simulink model "Dinamica5seg"  (R2021b)
settings: Solver=VariableStepAuto  StartTime=0.0  StopTime=70  RelTol=1e-3
(part 2 of 3)

== matlab function Dinamica5seg/ROBOT ==
  data: q1 input; tao1 output; tao2 output; tao3 output; dq1 input; d2q1 input; q2 input; dq2 input; d2q2 input; q3 input; dq3 input; d2q3 input; q4 input; dq4 input; d2q4 input; m1 input; m2 input; m3 input; m4 input; l1 input; l2 input; l3 input; l4 input; g input; tao4 output
function [tao1, tao2, tao3, tao4] = EulerLagrange(q1, dq1, d2q1, q2, dq2, d2q2, q3, dq3, d2q3, q4, dq4, d2q4, m1, m2, m3, m4, l1, l2, l3, l4, g)
%tao1= (40812255641599999*d2q1)/16777216 - 999120000*dq2^2*cos(q1)^2 + 382320000*dq3^2*cos(q1)^2 + 191160000*dq3^2*cos(q2)^2 - 120720000*dq4^2*cos(q2)^2 + 120720000*dq4^2*cos(q3)^2 + (52562346639359997*dq2^2*sin(2*q1))/67108864 - (4500767812266667*dq3^2*sin(2*q1))/67108864 + 233160000*d2q2*cos(q1) + (9002430409386667*d2q3*cos(q2))/16777216 + 499560000*dq2^2 - 191160000*dq3^2 - (13504093006506667*dq2*dq3*sin(q2))/33554432 + 80480000*d2q4*cos(q1)*cos(q3) - 382320000*dq3^2*cos(q1)^2*cos(q2)^2 + 241440000*dq4^2*cos(q1)^2*cos(q2)^2 - 241440000*dq4^2*cos(q1)^2*cos(q3)^2 + 120720000*dq4^2*cos(q2)^2*cos(q3)^2 + 150920000*d2q3*sin(q1)*sin(q2) + (5850998155946667*d2q4*sin(q2)*sin(q3))/16777216 + d2q1*l1^2*m1 + (d2q1*l1^2*m2)/2 + (d2q1*l1^2*m3)/2 + (d2q1*l1^2*m4)/2 + (d2q1*l3^2*m3)/8 + (d2q1*l3^2*m4)/2 + (d2q1*l4^2*m4)/8 + 241440000*dq2*dq4*cos(q3) + (4500767812266667*dq3^2*cos(q1)*cos(q2)^2*sin(q1))/33554432 - (4500767812266667*dq4^2*cos(q1)*cos(q2)^2*sin(q1))/33554432 + (4500767812266667*dq4^2*cos(q1)*cos(q3)^2*sin(q1))/33554432 + (d2q1*l2^2*m2*cos(q2)^2)/8 + (d2q1*l2^2*m3*cos(q2)^2)/2 + (d2q1*l2^2*m4*cos(q2)^2)/2 - (d2q1*l3^2*m3*cos(q3)^2)/8 - (d2q1*l3^2*m4*cos(q3)^2)/2 - (d2q1*l4^2*m4*cos(q2)^2)/8 - 482880000*dq2*dq4*cos(q1)^2*cos(q3) - (4500767812266667*dq2*dq3*cos(q1)^2*sin(q2))/16777216 - 80480000*d2q4*cos(q2)*sin(q1)*sin(q3) + (g*l1*m1*cos(q1))/2 + g*l1*m2*cos(q1) + g*l1*m3*cos(q1) + g*l1*m4*cos(q1) - 150920000*dq3^2*cos(q1)*cos(q2)*sin(q2) + 80480000*dq4^2*cos(q1)*cos(q2)*sin(q2) - (4500767812266667*dq4^2*cos(q2)*cos(q3)*sin(q3))/33554432 - 241440000*dq4^2*cos(q1)^2*cos(q2)^2*cos(q3)^2 + (d2q3*l3^2*m3*cos(q2))/8 + (d2q3*l3^2*m4*cos(q2))/2 + 301840000*dq2*dq3*cos(q2)*sin(q1) + (7201228499626667*dq2*dq4*cos(q2)*sin(q3))/33554432 - 160960000*dq3*dq4*cos(q1)*sin(q3) + (16202764124160001*dq3*dq4*cos(q3)*sin(q2))/33554432 + (d2q3*l4^2*m4*cos(q2)*cos(q4)^2)/8 + (4500767812266667*dq2*dq4*cos(q1)^2*cos(q2)*sin(q3))/16777216 + 160960000*dq3*dq4*cos(q1)*cos(q2)^2*sin(q3) - (4500767812266667*dq3*dq4*cos(q1)^2*cos(q3)*sin(q2))/16777216 + (4500767812266667*dq4^2*cos(q1)*cos(q2)^2*cos(q3)^2*sin(q1))/33554432 - (dq2*dq3*l3^2*m3*sin(q2))/4 - dq2*dq3*l3^2*m4*sin(q2) + (g*l2*m2*cos(q1)*cos(q2))/2 + g*l2*m3*cos(q1)*cos(q2) + g*l2*m4*cos(q1)*cos(q2) - (dq3^2*l1*l3*m3*sin(q3))/4 - (dq3^2*l1*l3*m4*sin(q3))/2 + (d2q1*l3^2*m3*cos(q2)^2*cos(q3)^2)/8 + (d2q1*l3^2*m4*cos(q2)^2*cos(q3)^2)/2 + (d2q1*l4^2*m4*cos(q2)^2*cos(q4)^2)/8 - (d2q1*l4^2*m4*cos(q3)^2*cos(q4)^2)/8 - (g*l3*m3*sin(q1)*sin(q3))/2 - g*l3*m4*sin(q1)*sin(q3) - (dq1*dq2*l2^2*m2*sin(2*q2))/8 - (dq1*dq2*l2^2*m3*sin(2*q2))/2 - (dq1*dq2*l2^2*m4*sin(2*q2))/2 + (dq1*dq2*l4^2*m4*sin(2*q2))/8 + (dq1*dq3*l3^2*m3*sin(2*q3))/8 + (dq1*dq3*l3^2*m4*sin(2*q3))/2 + 80480000*dq4^2*cos(q3)*sin(q1)*sin(q2)*sin(q3) + (4500767812266667*dq2*dq4*cos(q1)*cos(q3)*sin(q1))/16777216 + (d2q4*l4^2*m4*sin(q2)*sin(q3))/8 - 764640000*dq2*dq3*cos(q1)*sin(q1)*sin(q2) + 241440000*dq3*dq4*cos(q2)*sin(q2)*sin(q3) + 160960000*dq2*dq4*sin(q1)*sin(q2)*sin(q3) + (d2q1*l1*l2*m2*cos(q2))/2 + d2q1*l1*l2*m3*cos(q2) + d2q1*l1*l2*m4*cos(q2) + (d2q3*l1*l3*m3*cos(q3))/4 + (d2q3*l1*l3*m4*cos(q3))/2 + (d2q1*l3*l4*m4*cos(q4))/2 - 80480000*dq4^2*cos(q1)*cos(q2)*cos(q3)^2*sin(q2) + (4500767812266667*dq4^2*cos(q1)^2*cos(q2)*cos(q3)*sin(q3))/16777216 + (d2q1*l2*l3*m3*cos(q2)^2*cos(q3))/2 + d2q1*l2*l3*m4*cos(q2)^2*cos(q3) - (d2q1*l3*l4*m4*cos(q3)^2*cos(q4))/2 + (dq3*dq4*l4^2*m4*cos(q3)*sin(q2))/4 + (g*l3*m3*cos(q1)*cos(q2)*cos(q3))/2 + g*l3*m4*cos(q1)*cos(q2)*cos(q3) + (dq2^2*l2*l3*m3*cos(q2)*sin(q3))/4 + (dq2^2*l2*l3*m4*cos(q2)*sin(q3))/2 - (dq3^2*l2*l3*m3*cos(q2)*sin(q3))/4 - (dq3^2*l2*l3*m4*cos(q2)*sin(q3))/2 - (dq3^2*l1*l4*m4*cos(q4)*sin(q3))/4 - (dq4^2*l1*l4*m4*cos(q4)*sin(q3))/4 - (g*l4*m4*cos(q1)*sin(q2)*sin(q4))/2 - (g*l4*m4*cos(q4)*sin(q1)*sin(q3))/2 - (dq1*dq2*l1*l2*m2*sin(q2))/2 - dq1*dq2*l1*l2*m3*sin(q2) - dq1*dq2*l1*l2*m4*sin(q2) + (dq1*dq2*l2*l4*m4*sin(q4))/2 - (dq1*dq4*l3*l4*m4*sin(q4))/2 + 482880000*dq4^2*cos(q1)*cos(q2)*cos(q3)*sin(q1)*sin(q3) + (dq2*dq3*l3^2*m3*cos(q3)^2*sin(q2))/4 + dq2*dq3*l3^2*m4*cos(q3)^2*sin(q2) - (dq2*dq3*l4^2*m4*cos(q4)^2*sin(q2))/4 + (d2q1*l4^2*m4*cos(q2)^2*cos(q3)^2*cos(q4)^2)/8 + (d2q2*l3^2*m3*cos(q3)*sin(q2)*sin(q3))/8 + (d2q2*l3^2*m4*cos(q3)*sin(q2)*sin(q3))/2 + 482880000*dq2*dq4*cos(q1)*cos(q2)*sin(q1)*sin(q3) - 482880000*dq3*dq4*cos(q1)*cos(q3)*sin(q1)*sin(q2) + (d2q1*l1*l3*m3*cos(q2)*cos(q3))/2 + d2q1*l1*l3*m4*cos(q2)*cos(q3) + (d2q3*l2*l3*m3*cos(q2)*cos(q3))/4 + (d2q3*l2*l3*m4*cos(q2)*cos(q3))/2 + (d2q3*l1*l4*m4*cos(q3)*cos(q4))/4 + (d2q3*l3*l4*m4*cos(q2)*cos(q4))/2 + (d2q2*l2*l3*m3*sin(q2)*sin(q3))/4 - (d2q1*l1*l4*m4*sin(q2)*sin(q4))/2 + (d2q2*l2*l3*m4*sin(q2)*sin(q3))/2 - (d2q4*l1*l4*m4*sin(q3)*sin(q4))/4 + (dq2^2*l3^2*m3*cos(q2)*cos(q3)*sin(q3))/8 + (dq2^2*l3^2*m4*cos(q2)*cos(q3)*sin(q3))/2 - 482880000*dq3*dq4*cos(q1)^2*cos(q2)*sin(q2)*sin(q3) - (dq2^2*l3*l4*m4*sin(q2)*sin(q3)*sin(q4))/4 + (dq3^2*l3*l4*m4*sin(q2)*sin(q3)*sin(q4))/4 - (dq4^2*l3*l4*m4*sin(q2)*sin(q3)*sin(q4))/4 + (dq2^2*l4^2*m4*cos(q2)*cos(q3)*cos(q4)^2*sin(q3))/8 - (dq1*dq2*l1*l3*m3*cos(q3)*sin(q2))/2 - dq1*dq2*l1*l3*m4*cos(q3)*sin(q2) - (dq1*dq3*l1*l3*m3*cos(q2)*sin(q3))/2 - dq1*dq3*l1*l3*m4*cos(q2)*sin(q3) - (dq1*dq2*l1*l4*m4*cos(q2)*sin(q4))/2 - (dq1*dq4*l1*l4*m4*cos(q4)*sin(q2))/2 + (dq1*dq2*l3*l4*m4*cos(q3)*sin(q4))/2 - dq2*dq3*l3*l4*m4*cos(q4)*sin(q2) - (dq3*dq4*l1*l4*m4*cos(q3)*sin(q4))/2 - (dq3*dq4*l3*l4*m4*cos(q2)*sin(q4))/2 + (d2q1*l3*l4*m4*cos(q2)^2*cos(q3)^2*cos(q4))/2 - (dq1*dq2*l3^2*m3*cos(q2)*cos(q3)^2*sin(q2))/4 - dq1*dq2*l3^2*m4*cos(q2)*cos(q3)^2*sin(q2) - (dq1*dq3*l3^2*m3*cos(q2)^2*cos(q3)*sin(q3))/4 - (dq1*dq2*l4^2*m4*cos(q2)*cos(q4)^2*sin(q2))/4 - dq1*dq3*l3^2*m4*cos(q2)^2*cos(q3)*sin(q3) + (dq1*dq3*l4^2*m4*cos(q3)*cos(q4)^2*sin(q3))/4 - (dq1*dq4*l4^2*m4*cos(q2)^2*cos(q4)*sin(q4))/4 + (dq2*dq4*l4^2*m4*cos(q2)*cos(q4)^2*sin(q3))/4 + (dq1*dq4*l4^2*m4*cos(q3)^2*cos(q4)*sin(q4))/4 - (dq3*dq4*l4^2*m4*cos(q3)*cos(q4)^2*sin(q2))/4 + (d2q2*l4^2*m4*cos(q2)*cos(q4)*sin(q3)*sin(q4))/8 - (d2q3*l4^2*m4*cos(q3)*cos(q4)*sin(q2)*sin(q4))/8 + (4500767812266667*dq3*dq4*cos(q1)*cos(q2)*sin(q1)*sin(q2)*sin(q3))/16777216 - (dq1*dq3*l2*l3*m3*cos(q2)^2*sin(q3))/2 - dq1*dq3*l2*l3*m4*cos(q2)^2*sin(q3) - dq1*dq2*l2*l4*m4*cos(q2)^2*sin(q4) + (dq1*dq4*l3*l4*m4*cos(q3)^2*sin(q4))/2 + (d2q1*l1*l4*m4*cos(q2)*cos(q3)*cos(q4))/2 + (d2q3*l2*l4*m4*cos(q2)*cos(q3)*cos(q4))/4 - (d2q1*l2*l4*m4*cos(q2)*sin(q2)*sin(q4))/2 + (d2q2*l2*l4*m4*cos(q4)*sin(q2)*sin(q3))/4 + (d2q2*l3*l4*m4*cos(q2)*sin(q3)*sin(q4))/4 - (d2q3*l3*l4*m4*cos(q3)*sin(q2)*sin(q4))/4 - (d2q4*l2*l4*m4*cos(q2)*sin(q3)*sin(q4))/4 + (d2q4*l3*l4*m4*cos(q4)*sin(q2)*sin(q3))/4 + (dq2*dq3*l4^2*m4*cos(q3)^2*cos(q4)^2*sin(q2))/4 + (d2q2*l4^2*m4*cos(q3)*cos(q4)^2*sin(q2)*sin(q3))/8 - (dq2^2*l4^2*m4*cos(q4)*sin(q2)*sin(q3)*sin(q4))/8 + (dq3^2*l4^2*m4*cos(q4)*sin(q2)*sin(q3)*sin(q4))/8 + (d2q1*l2*l4*m4*cos(q2)^2*cos(q3)*cos(q4))/2 + (dq1*dq4*l4^2*m4*cos(q2)*cos(q3)*sin(q2))/4 + (dq1*dq2*l4^2*m4*cos(q3)*cos(q4)*sin(q4))/4 - (dq3*dq4*l4^2*m4*cos(q2)*cos(q4)*sin(q4))/4 + (g*l4*m4*cos(q1)*cos(q2)*cos(q3)*cos(q4))/2 + (dq2^2*l2*l4*m4*cos(q2)*cos(q4)*sin(q3))/4 - (dq3^2*l2*l4*m4*cos(q2)*cos(q4)*sin(q3))/4 - (dq4^2*l2*l4*m4*cos(q2)*cos(q4)*sin(q3))/4 - (dq1*dq2*l4^2*m4*cos(q2)^2*cos(q3)*cos(q4)*sin(q4))/2 - (dq1*dq4*l4^2*m4*cos(q2)*cos(q3)*cos(q4)^2*sin(q2))/2 - (d2q1*l4^2*m4*cos(q2)*cos(q3)*cos(q4)*sin(q2)*sin(q4))/4 - dq1*dq2*l3*l4*m4*cos(q2)^2*cos(q3)*sin(q4) - (dq1*dq3*l2*l4*m4*cos(q2)^2*cos(q4)*sin(q3))/2 - (dq1*dq4*l2*l4*m4*cos(q2)^2*cos(q3)*sin(q4))/2 + dq2*dq3*l3*l4*m4*cos(q3)^2*cos(q4)*sin(q2) - (d2q1*l3*l4*m4*cos(q2)*cos(q3)*sin(q2)*sin(q4))/2 + (d2q2*l3*l4*m4*cos(q3)*cos(q4)*sin(q2)*sin(q3))/2 - (dq1*dq2*l4^2*m4*cos(q2)*cos(q3)^2*cos(q4)^2*sin(q2))/4 - (dq1*dq3*l4^2*m4*cos(q2)^2*cos(q3)*cos(q4)^2*sin(q3))/4 - (dq1*dq4*l4^2*m4*cos(q2)^2*cos(q3)^2*cos(q4)*sin(q4))/4 - (dq1*dq4*l3*l4*m4*cos(q2)^2*cos(q3)^2*sin(q4))/2 + (dq2^2*l3*l4*m4*cos(q2)*cos(q3)*cos(q4)*sin(q3))/2 - dq1*dq2*l2*l3*m3*cos(q2)*cos(q3)*sin(q2) - 2*dq1*dq2*l2*l3*m4*cos(q2)*cos(q3)*sin(q2) - (dq1*dq2*l1*l4*m4*cos(q3)*cos(q4)*sin(q2))/2 - (dq1*dq3*l1*l4*m4*cos(q2)*cos(q4)*sin(q3))/2 - (dq1*dq4*l1*l4*m4*cos(q2)*cos(q3)*sin(q4))/2 - (dq1*dq4*l2*l4*m4*cos(q2)*cos(q4)*sin(q2))/2 + dq1*dq3*l3*l4*m4*cos(q3)*cos(q4)*sin(q3) + (dq2*dq4*l3*l4*m4*cos(q2)*cos(q4)*sin(q3))/2 - (dq3*dq4*l2*l4*m4*cos(q2)*cos(q3)*sin(q4))/2 - dq1*dq2*l3*l4*m4*cos(q2)*cos(q3)^2*cos(q4)*sin(q2) - dq1*dq3*l3*l4*m4*cos(q2)^2*cos(q3)*cos(q4)*sin(q3) + (dq1*dq3*l4^2*m4*cos(q2)*cos(q4)*sin(q2)*sin(q3)*sin(q4))/4 - (dq2*dq4*l4^2*m4*cos(q3)*cos(q4)*sin(q2)*sin(q3)*sin(q4))/4 - dq1*dq2*l2*l4*m4*cos(q2)*cos(q3)*cos(q4)*sin(q2) - (dq1*dq4*l3*l4*m4*cos(q2)*cos(q3)*cos(q4)*sin(q2))/2 + (dq1*dq3*l3*l4*m4*cos(q2)*sin(q2)*sin(q3)*sin(q4))/2 - (dq2*dq4*l3*l4*m4*cos(q3)*sin(q2)*sin(q3)*sin(q4))/2;
%tao2= (20862803640320001*d2q2)/33554432 + 499560000*d2q2*sin(2*q1) - 233160000*dq1^2*sin(q1) + 150920000*dq3^2*sin(q1) - 80480000*dq4^2*sin(q1) - 999120000*dq1*dq2 + 233160000*d2q1*cos(q1) + (7201228499626667*d2q4*cos(q3))/33554432 + 191160000*d2q3*sin(q2) + (52562346639359997*d2q2*cos(q1)^2)/33554432 + (13504093006506667*dq1*dq3*sin(q2))/33554432 - (7201228499626667*dq3*dq4*sin(q3))/33554432 - 301840000*dq3^2*cos(q2)^2*sin(q1) + 160960000*dq4^2*cos(q2)^2*sin(q1) + 80480000*dq4^2*cos(q3)^2*sin(q1) + 1998240000*dq1*dq2*cos(q1)^2 - (52562346639359997*dq1*dq2*sin(2*q1))/33554432 + 150920000*d2q3*cos(q1)*cos(q2) - 120720000*d2q4*cos(q2)*sin(q3) + (4500767812266667*d2q4*cos(q1)^2*cos(q3))/33554432 - 382320000*d2q3*cos(q1)^2*sin(q2) + (d2q2*l2^2*m2)/8 + (d2q2*l2^2*m3)/2 + (d2q2*l2^2*m4)/2 + (d2q2*l4^2*m4)/8 - 241440000*dq1*dq4*cos(q3) + (4500767812266667*dq3^2*cos(q1)^2*cos(q2)*sin(q2))/33554432 - (4500767812266667*dq4^2*cos(q1)^2*cos(q2)*sin(q2))/33554432 + (d2q2*l3^2*m3*cos(q3)^2)/8 + (d2q2*l3^2*m4*cos(q3)^2)/2 - (d2q2*l4^2*m4*cos(q4)^2)/8 + 482880000*dq1*dq4*cos(q1)^2*cos(q3) + (4500767812266667*dq1*dq3*cos(q1)^2*sin(q2))/16777216 + 241440000*d2q4*cos(q1)*cos(q3)*sin(q1) + (4500767812266667*d2q3*cos(q1)*sin(q1)*sin(q2))/33554432 + 80480000*d2q4*cos(q1)*sin(q2)*sin(q3) - 160960000*dq4^2*cos(q2)^2*cos(q3)^2*sin(q1) + (dq1^2*l2^2*m2*sin(2*q2))/16 + (dq1^2*l2^2*m3*sin(2*q2))/4 + (dq1^2*l2^2*m4*sin(2*q2))/4 - (dq1^2*l4^2*m4*sin(2*q2))/16 + 241440000*d2q4*cos(q1)^2*cos(q2)*sin(q3) - 120720000*dq4^2*cos(q3)*sin(q2)*sin(q3) + (d2q4*l4^2*m4*cos(q3))/8 - 241440000*dq3*dq4*cos(q2)*cos(q3) - 301840000*dq1*dq3*cos(q2)*sin(q1) - (7201228499626667*dq1*dq4*cos(q2)*sin(q3))/33554432 + 482880000*dq3*dq4*cos(q1)^2*cos(q2)*cos(q3) - (4500767812266667*dq1*dq4*cos(q1)^2*cos(q2)*sin(q3))/16777216 - (4500767812266667*d2q4*cos(q1)*cos(q2)*sin(q1)*sin(q3))/33554432 + (4500767812266667*dq4^2*cos(q1)^2*cos(q2)*cos(q3)^2*sin(q2))/33554432 - (dq3*dq4*l4^2*m4*sin(q3))/4 + (dq1^2*l1*l2*m2*sin(q2))/4 + (dq1^2*l1*l2*m3*sin(q2))/2 + (dq1^2*l1*l2*m4*sin(q2))/2 - (dq1^2*l2*l4*m4*sin(q4))/4 - (dq4^2*l2*l4*m4*sin(q4))/4 + (d2q2*l4^2*m4*cos(q3)^2*cos(q4)^2)/8 - (g*l2*m2*sin(q1)*sin(q2))/2 - g*l2*m3*sin(q1)*sin(q2) - g*l2*m4*sin(q1)*sin(q2) - (4500767812266667*dq3*dq4*cos(q1)^2*cos(q2)^2*sin(q3))/16777216 - 80480000*dq4^2*cos(q1)*cos(q2)*cos(q3)*sin(q3) + 382320000*dq3^2*cos(q1)*cos(q2)*sin(q1)*sin(q2) - 241440000*dq4^2*cos(q1)*cos(q2)*sin(q1)*sin(q2) - (dq2*dq3*l3^2*m3*sin(2*q3))/8 - (dq2*dq3*l3^2*m4*sin(2*q3))/2 + (dq2*dq4*l4^2*m4*sin(2*q4))/8 - (4500767812266667*dq1*dq4*cos(q1)*cos(q3)*sin(q1))/16777216 + 160960000*dq3*dq4*cos(q1)*cos(q3)*sin(q2) + 764640000*dq1*dq3*cos(q1)*sin(q1)*sin(q2) - 160960000*dq1*dq4*sin(q1)*sin(q2)*sin(q3) + (d2q2*l2*l3*m3*cos(q3))/2 + d2q2*l2*l3*m4*cos(q3) + (d2q4*l2*l4*m4*cos(q4))/4 + 241440000*dq4^2*cos(q1)^2*cos(q3)*sin(q2)*sin(q3) + (d2q2*l3*l4*m4*cos(q3)^2*cos(q4))/2 - (dq1*dq4*l4^2*m4*cos(q2)*sin(q3))/4 + (dq1^2*l1*l3*m3*cos(q3)*sin(q2))/4 + (dq1^2*l1*l3*m4*cos(q3)*sin(q2))/2 + (dq1^2*l1*l4*m4*cos(q2)*sin(q4))/4 - (dq1^2*l3*l4*m4*cos(q3)*sin(q4))/4 + (dq3^2*l3*l4*m4*cos(q3)*sin(q4))/4 - (dq4^2*l3*l4*m4*cos(q3)*sin(q4))/4 - (g*l3*m3*cos(q3)*sin(q1)*sin(q2))/2 - g*l3*m4*cos(q3)*sin(q1)*sin(q2) - (g*l4*m4*cos(q2)*sin(q1)*sin(q4))/2 + (dq1^2*l3^2*m3*cos(q2)*cos(q3)^2*sin(q2))/8 + (dq1^2*l3^2*m4*cos(q2)*cos(q3)^2*sin(q2))/2 + (dq1^2*l4^2*m4*cos(q2)*cos(q4)^2*sin(q2))/8 - (dq2*dq3*l2*l3*m3*sin(q3))/2 - dq2*dq3*l2*l3*m4*sin(q3) + (dq1*dq3*l3^2*m3*cos(q3)^2*sin(q2))/4 + dq1*dq3*l3^2*m4*cos(q3)^2*sin(q2) + (dq3*dq4*l4^2*m4*cos(q4)^2*sin(q3))/4 - (4500767812266667*dq4^2*cos(q1)*cos(q3)*sin(q1)*sin(q2)*sin(q3))/33554432 + (dq1^2*l2*l4*m4*cos(q2)^2*sin(q4))/2 - (4500767812266667*dq3*dq4*cos(q1)*cos(q2)*cos(q3)*sin(q1))/16777216 + (d2q1*l3^2*m3*cos(q3)*sin(q2)*sin(q3))/8 + (d2q1*l3^2*m4*cos(q3)*sin(q2)*sin(q3))/2 + (d2q3*l4^2*m4*cos(q4)*sin(q3)*sin(q4))/8 - 482880000*dq1*dq4*cos(q1)*cos(q2)*sin(q1)*sin(q3) - 321920000*dq3*dq4*cos(q2)*sin(q1)*sin(q2)*sin(q3) + (d2q2*l2*l4*m4*cos(q3)*cos(q4))/2 + (d2q4*l3*l4*m4*cos(q3)*cos(q4))/4 + 241440000*dq4^2*cos(q1)*cos(q2)*cos(q3)^2*sin(q1)*sin(q2) + (d2q1*l2*l3*m3*sin(q2)*sin(q3))/4 + (d2q1*l2*l3*m4*sin(q2)*sin(q3))/2 + (d2q3*l3*l4*m4*sin(q3)*sin(q4))/4 - (dq1^2*l4^2*m4*cos(q3)*cos(q4)*sin(q4))/8 + (dq3^2*l4^2*m4*cos(q3)*cos(q4)*sin(q4))/8 - 482880000*dq3*dq4*cos(q1)*cos(q2)^2*sin(q1)*sin(q3) - (g*l4*m4*cos(q3)*cos(q4)*sin(q1)*sin(q2))/2 + (dq1^2*l4^2*m4*cos(q2)^2*cos(q3)*cos(q4)*sin(q4))/4 + (dq1*dq3*l2*l3*m3*cos(q3)*sin(q2))/2 + dq1*dq3*l2*l3*m4*cos(q3)*sin(q2) - (dq2*dq3*l2*l4*m4*cos(q4)*sin(q3))/2 - (dq2*dq4*l2*l4*m4*cos(q3)*sin(q4))/2 + (dq1*dq4*l4^2*m4*cos(q2)*cos(q4)^2*sin(q3))/4 - (dq2*dq3*l4^2*m4*cos(q3)*cos(q4)^2*sin(q3))/4 - (dq2*dq4*l4^2*m4*cos(q3)^2*cos(q4)*sin(q4))/4 + (dq1^2*l3*l4*m4*cos(q2)^2*cos(q3)*sin(q4))/2 + (d2q1*l4^2*m4*cos(q2)*cos(q4)*sin(q3)*sin(q4))/8 + (dq1^2*l4^2*m4*cos(q2)*cos(q3)^2*cos(q4)^2*sin(q2))/8 - (dq2*dq4*l3*l4*m4*cos(q3)^2*sin(q4))/2 + (d2q1*l2*l4*m4*cos(q4)*sin(q2)*sin(q3))/4 + (d2q1*l3*l4*m4*cos(q2)*sin(q3)*sin(q4))/4 + (dq1*dq3*l4^2*m4*cos(q3)^2*cos(q4)^2*sin(q2))/4 + (d2q1*l4^2*m4*cos(q3)*cos(q4)^2*sin(q2)*sin(q3))/8 + (dq1^2*l2*l3*m3*cos(q2)*cos(q3)*sin(q2))/2 + dq1^2*l2*l3*m4*cos(q2)*cos(q3)*sin(q2) + (dq1^2*l1*l4*m4*cos(q3)*cos(q4)*sin(q2))/4 - (dq1*dq4*l2*l4*m4*sin(q2)*sin(q3)*sin(q4))/2 + (dq1^2*l3*l4*m4*cos(q2)*cos(q3)^2*cos(q4)*sin(q2))/2 + dq1*dq3*l3*l4*m4*cos(q3)^2*cos(q4)*sin(q2) + (d2q1*l3*l4*m4*cos(q3)*cos(q4)*sin(q2)*sin(q3))/2 + (dq1*dq3*l4^2*m4*cos(q2)*cos(q3)*cos(q4)*sin(q4))/4 + (dq1^2*l2*l4*m4*cos(q2)*cos(q3)*cos(q4)*sin(q2))/2 + (dq1*dq3*l2*l4*m4*cos(q3)*cos(q4)*sin(q2))/2 + (dq1*dq3*l3*l4*m4*cos(q2)*cos(q3)*sin(q4))/2 - dq2*dq3*l3*l4*m4*cos(q3)*cos(q4)*sin(q3) - (dq1*dq4*l4^2*m4*cos(q3)*cos(q4)*sin(q2)*sin(q3)*sin(q4))/4 - (dq1*dq4*l3*l4*m4*cos(q3)*sin(q2)*sin(q3)*sin(q4))/2;
%tao3= (9002430409386667*d2q3)/16777216 - 191160000*d2q3*sin(2*q1) + 382320000*dq1*dq3 - (4500767812266667*dq4^2*sin(2*q3))/67108864 + (9002430409386667*d2q1*cos(q2))/16777216 + 191160000*d2q2*sin(q2) - (4500767812266667*d2q3*cos(q1)^2)/33554432 + 191160000*dq2^2*cos(q2) - 120720000*dq4^2*cos(q2) - (22505628631040001*dq1*dq2*sin(q2))/33554432 - 301840000*dq2*dq3*sin(q1) + (7201228499626667*dq2*dq4*sin(q3))/33554432 + (4500767812266667*d2q3*cos(q1)^2*cos(q2)^2)/33554432 - 382320000*dq2^2*cos(q1)^2*cos(q2) + 241440000*dq4^2*cos(q1)^2*cos(q2) + 241440000*dq4^2*cos(q2)*cos(q3)^2 - 764640000*dq1*dq3*cos(q1)^2 - 382320000*dq1*dq3*cos(q2)^2 + (4500767812266667*dq1*dq3*sin(2*q1))/33554432 + 150920000*d2q2*cos(q1)*cos(q2) + 120720000*d2q4*cos(q3)*sin(q2) + 150920000*d2q1*sin(q1)*sin(q2) + 80480000*d2q4*sin(q1)*sin(q3) - 382320000*d2q2*cos(q1)^2*sin(q2) + 150920000*dq1^2*cos(q1)*sin(q2) - 150920000*dq2^2*cos(q1)*sin(q2) + 80480000*dq4^2*cos(q1)*sin(q2) + (d2q3*l3^2*m3)/8 + (d2q3*l3^2*m4)/2 - 160960000*dq4^2*cos(q1)*cos(q3)^2*sin(q2) + (4500767812266667*dq4^2*cos(q1)^2*cos(q3)*sin(q3))/33554432 + (d2q3*l4^2*m4*cos(q4)^2)/8 + (4500767812266667*dq1*dq2*cos(q1)^2*sin(q2))/16777216 + 603680000*dq2*dq3*cos(q2)^2*sin(q1) + 80480000*d2q4*cos(q1)*cos(q2)*cos(q3) - 482880000*dq4^2*cos(q1)^2*cos(q2)*cos(q3)^2 + (4500767812266667*d2q2*cos(q1)*sin(q1)*sin(q2))/33554432 + 301840000*d2q3*cos(q2)*sin(q1)*sin(q2) + 764640000*dq1*dq3*cos(q1)^2*cos(q2)^2 - (dq1^2*l3^2*m3*sin(2*q3))/16 - (dq1^2*l3^2*m4*sin(2*q3))/4 + (dq2^2*l3^2*m3*sin(2*q3))/16 + (dq2^2*l3^2*m4*sin(2*q3))/4 + 382320000*d2q3*cos(q1)*cos(q2)^2*sin(q1) - 241440000*d2q4*cos(q1)^2*cos(q3)*sin(q2) + (4500767812266667*dq2^2*cos(q1)*cos(q2)*sin(q1))/33554432 - (4500767812266667*dq4^2*cos(q1)*cos(q2)*sin(q1))/33554432 - 160960000*d2q4*cos(q2)^2*sin(q1)*sin(q3) + (d2q1*l3^2*m3*cos(q2))/8 + (d2q1*l3^2*m4*cos(q2))/2 + 241440000*dq2*dq4*cos(q2)*cos(q3) + 160960000*dq1*dq4*cos(q1)*sin(q3) - (16202764124160001*dq1*dq4*cos(q3)*sin(q2))/33554432 + (d2q1*l4^2*m4*cos(q2)*cos(q4)^2)/8 - 482880000*dq2*dq4*cos(q1)^2*cos(q2)*cos(q3) - (4500767812266667*dq1*dq3*cos(q1)*cos(q2)^2*sin(q1))/16777216 - (4500767812266667*dq2*dq3*cos(q1)^2*cos(q2)*sin(q2))/16777216 - 160960000*dq1*dq4*cos(q1)*cos(q2)^2*sin(q3) + (4500767812266667*dq1*dq4*cos(q1)^2*cos(q3)*sin(q2))/16777216 + (4500767812266667*d2q4*cos(q1)*cos(q3)*sin(q1)*sin(q2))/33554432 + (4500767812266667*dq4^2*cos(q1)^2*cos(q2)^2*cos(q3)*sin(q3))/33554432 + (g*l3*m3*cos(q1)*cos(q3))/2 + g*l3*m4*cos(q1)*cos(q3) + (dq2^2*l2*l3*m3*sin(q3))/4 + (dq2^2*l2*l3*m4*sin(q3))/2 + (4500767812266667*dq2*dq4*cos(q1)^2*cos(q2)^2*sin(q3))/16777216 + (4500767812266667*d2q4*cos(q1)^2*cos(q2)*sin(q2)*sin(q3))/33554432 + 241440000*dq4^2*cos(q1)*cos(q3)*sin(q1)*sin(q3) - (dq3*dq4*l4^2*m4*sin(2*q4))/8 + 301840000*dq1*dq3*cos(q1)*cos(q2)*sin(q2) - 160960000*dq2*dq4*cos(q1)*cos(q3)*sin(q2) + 764640000*dq1*dq2*cos(q1)*sin(q1)*sin(q2) - 241440000*dq1*dq4*cos(q2)*sin(q2)*sin(q3) + (d2q1*l1*l3*m3*cos(q3))/4 + (d2q1*l1*l3*m4*cos(q3))/2 + (d2q3*l3*l4*m4*cos(q4))/2 + (4500767812266667*dq4^2*cos(q1)*cos(q2)*cos(q3)^2*sin(q1))/16777216 + 241440000*d2q4*cos(q1)*cos(q2)*sin(q1)*sin(q2)*sin(q3) + (g*l4*m4*cos(q1)*cos(q3)*cos(q4))/2 + (dq1^2*l1*l3*m3*cos(q2)*sin(q3))/4 + (dq1^2*l1*l3*m4*cos(q2)*sin(q3))/2 + (dq2^2*l2*l4*m4*cos(q4)*sin(q3))/4 - (g*l3*m3*cos(q2)*sin(q1)*sin(q3))/2 - g*l3*m4*cos(q2)*sin(q1)*sin(q3) + (dq1^2*l3^2*m3*cos(q2)^2*cos(q3)*sin(q3))/8 + (dq1^2*l3^2*m4*cos(q2)^2*cos(q3)*sin(q3))/2 - (dq1^2*l4^2*m4*cos(q3)*cos(q4)^2*sin(q3))/8 + (dq2^2*l4^2*m4*cos(q3)*cos(q4)^2*sin(q3))/8 - (dq3*dq4*l3*l4*m4*sin(q4))/2 - (dq1*dq2*l3^2*m3*cos(q3)^2*sin(q2))/4 - dq1*dq2*l3^2*m4*cos(q3)^2*sin(q2) + (dq2*dq4*l4^2*m4*cos(q4)^2*sin(q3))/4 + 160960000*dq4^2*cos(q2)*cos(q3)*sin(q1)*sin(q2)*sin(q3) + (dq1^2*l2*l3*m3*cos(q2)^2*sin(q3))/4 + (dq1^2*l2*l3*m4*cos(q2)^2*sin(q3))/2 + (4500767812266667*dq2*dq4*cos(q1)*cos(q2)*cos(q3)*sin(q1))/16777216 + (d2q2*l4^2*m4*cos(q4)*sin(q3)*sin(q4))/8 - 764640000*dq2*dq3*cos(q1)*cos(q2)*sin(q1)*sin(q2) + 482880000*dq1*dq4*cos(q1)*cos(q3)*sin(q1)*sin(q2) + 321920000*dq2*dq4*cos(q2)*sin(q1)*sin(q2)*sin(q3) + (d2q1*l2*l3*m3*cos(q2)*cos(q3))/4 + (d2q1*l2*l3*m4*cos(q2)*cos(q3))/2 + (d2q1*l1*l4*m4*cos(q3)*cos(q4))/4 + (d2q1*l3*l4*m4*cos(q2)*cos(q4))/2 + 241440000*dq4^2*cos(q1)*cos(q2)^2*cos(q3)*sin(q1)*sin(q3) + (d2q2*l3*l4*m4*sin(q3)*sin(q4))/4 + 482880000*dq1*dq4*cos(q1)^2*cos(q2)*sin(q2)*sin(q3) + 482880000*dq2*dq4*cos(q1)*cos(q2)^2*sin(q1)*sin(q3) - (g*l4*m4*cos(q2)*cos(q4)*sin(q1)*sin(q3))/2 - (dq1*dq2*l2*l3*m3*cos(q3)*sin(q2))/2 - dq1*dq2*l2*l3*m4*cos(q3)*sin(q2) - (dq1*dq4*l3*l4*m4*cos(q2)*sin(q4))/2 + (dq2*dq4*l3*l4*m4*cos(q4)*sin(q3))/2 - (dq1*dq4*l4^2*m4*cos(q3)*cos(q4)^2*sin(q2))/4 + (dq1^2*l2*l4*m4*cos(q2)^2*cos(q4)*sin(q3))/4 - (d2q1*l4^2*m4*cos(q3)*cos(q4)*sin(q2)*sin(q4))/8 + (dq1^2*l4^2*m4*cos(q2)^2*cos(q3)*cos(q4)^2*sin(q3))/8 - (4500767812266667*dq1*dq4*cos(q1)*cos(q2)*sin(q1)*sin(q2)*sin(q3))/16777216 + (d2q1*l2*l4*m4*cos(q2)*cos(q3)*cos(q4))/4 - (d2q1*l3*l4*m4*cos(q3)*sin(q2)*sin(q4))/4 - (dq1*dq2*l4^2*m4*cos(q3)^2*cos(q4)^2*sin(q2))/4 - (dq1*dq4*l4^2*m4*cos(q2)*cos(q4)*sin(q4))/4 + (dq1^2*l1*l4*m4*cos(q2)*cos(q4)*sin(q3))/4 - (dq1^2*l3*l4*m4*cos(q3)*cos(q4)*sin(q3))/2 + (dq2^2*l3*l4*m4*cos(q3)*cos(q4)*sin(q3))/2 + (dq1^2*l3*l4*m4*cos(q2)^2*cos(q3)*cos(q4)*sin(q3))/2 - dq1*dq2*l3*l4*m4*cos(q3)^2*cos(q4)*sin(q2) - (dq1^2*l4^2*m4*cos(q2)*cos(q4)*sin(q2)*sin(q3)*sin(q4))/8 - (dq1*dq2*l4^2*m4*cos(q2)*cos(q3)*cos(q4)*sin(q4))/4 - (dq1^2*l3*l4*m4*cos(q2)*sin(q2)*sin(q3)*sin(q4))/4 - (dq1*dq2*l2*l4*m4*cos(q3)*cos(q4)*sin(q2))/2 - (dq1*dq2*l3*l4*m4*cos(q2)*cos(q3)*sin(q4))/2 - (dq1*dq4*l3*l4*m4*cos(q3)*cos(q4)*sin(q2))/2;
%tao4= (5850998155946667*d2q4)/16777216 + (7201228499626667*d2q2*cos(q3))/33554432 - (4500767812266667*d2q4*cos(q3)^2)/33554432 + 160960000*dq2*dq4*sin(q1) - (7201228499626667*dq2*dq3*sin(q3))/33554432 - (4500767812266667*d2q4*cos(q1)^2*cos(q2)^2)/33554432 + (4500767812266667*d2q4*cos(q1)^2*cos(q3)^2)/33554432 + 241440000*dq1*dq4*cos(q2)^2 - 241440000*dq1*dq4*cos(q3)^2 + (4500767812266667*dq3*dq4*sin(2*q3))/33554432 + 80480000*d2q1*cos(q1)*cos(q3) - 120720000*d2q2*cos(q2)*sin(q3) + 120720000*d2q3*cos(q3)*sin(q2) + (5850998155946667*d2q1*sin(q2)*sin(q3))/16777216 + 80480000*d2q3*sin(q1)*sin(q3) + (4500767812266667*d2q2*cos(q1)^2*cos(q3))/33554432 - 80480000*dq1^2*cos(q3)*sin(q1) + 80480000*dq3^2*cos(q3)*sin(q1) + 120720000*dq2^2*sin(q2)*sin(q3) - 120720000*dq3^2*sin(q2)*sin(q3) + (d2q4*l4^2*m4)/8 - 241440000*dq1*dq2*cos(q3) + 241440000*dq3*dq4*cos(q2) - 160960000*dq3^2*cos(q2)^2*cos(q3)*sin(q1) - 241440000*dq2^2*cos(q1)^2*sin(q2)*sin(q3) + 241440000*dq3^2*cos(q1)^2*sin(q2)*sin(q3) + 482880000*dq1*dq2*cos(q1)^2*cos(q3) - 482880000*dq3*dq4*cos(q1)^2*cos(q2) - 482880000*dq3*dq4*cos(q2)*cos(q3)^2 - (4500767812266667*dq2*dq3*cos(q1)^2*sin(q3))/16777216 - 321920000*dq2*dq4*cos(q2)^2*sin(q1) - 160960000*dq2*dq4*cos(q3)^2*sin(q1) + 80480000*d2q3*cos(q1)*cos(q2)*cos(q3) + 241440000*d2q2*cos(q1)*cos(q3)*sin(q1) - 241440000*d2q4*cos(q2)*cos(q3)*sin(q3) + (4500767812266667*d2q4*cos(q1)^2*cos(q2)^2*cos(q3)^2)/33554432 - 80480000*d2q1*cos(q2)*sin(q1)*sin(q3) + 80480000*d2q2*cos(q1)*sin(q2)*sin(q3) - 160960000*d2q4*cos(q2)*sin(q1)*sin(q2) - 482880000*dq1*dq4*cos(q1)^2*cos(q2)^2 + 482880000*dq1*dq4*cos(q1)^2*cos(q3)^2 - 241440000*dq1*dq4*cos(q2)^2*cos(q3)^2 - (dq2^2*l4^2*m4*sin(2*q4))/16 + (dq3^2*l4^2*m4*sin(2*q4))/16 + 241440000*d2q2*cos(q1)^2*cos(q2)*sin(q3) - 241440000*d2q4*cos(q1)*cos(q2)^2*sin(q1) - 241440000*d2q3*cos(q1)^2*cos(q3)*sin(q2) + 241440000*d2q4*cos(q1)*cos(q3)^2*sin(q1) - 80480000*dq1^2*cos(q1)*cos(q2)*sin(q3) + 80480000*dq2^2*cos(q1)*cos(q2)*sin(q3) - 80480000*dq3^2*cos(q1)*cos(q2)*sin(q3) - 160960000*d2q3*cos(q2)^2*sin(q1)*sin(q3) + (d2q2*l4^2*m4*cos(q3))/8 + (16202764124160001*dq1*dq2*cos(q2)*sin(q3))/33554432 + (7201228499626667*dq1*dq3*cos(q3)*sin(q2))/33554432 - 160960000*dq3*dq4*cos(q1)*sin(q2) - (4500767812266667*dq1*dq2*cos(q1)^2*cos(q2)*sin(q3))/16777216 + (4500767812266667*dq1*dq4*cos(q1)*cos(q2)^2*sin(q1))/16777216 - 160960000*dq1*dq3*cos(q1)*cos(q2)^2*sin(q3) + (4500767812266667*dq1*dq3*cos(q1)^2*cos(q3)*sin(q2))/16777216 - (4500767812266667*dq1*dq4*cos(q1)*cos(q3)^2*sin(q1))/16777216 + (4500767812266667*dq2*dq4*cos(q1)^2*cos(q2)*sin(q2))/16777216 + 321920000*dq3*dq4*cos(q1)*cos(q3)^2*sin(q2) - (4500767812266667*dq3*dq4*cos(q1)^2*cos(q3)*sin(q3))/16777216 - (4500767812266667*d2q2*cos(q1)*cos(q2)*sin(q1)*sin(q3))/33554432 + (4500767812266667*d2q3*cos(q1)*cos(q3)*sin(q1)*sin(q2))/33554432 + 160960000*d2q4*cos(q1)*cos(q3)*sin(q2)*sin(q3) + (dq1^2*l3*l4*m4*sin(q4))/4 + (dq3^2*l3*l4*m4*sin(q4))/4 + 965760000*dq3*dq4*cos(q1)^2*cos(q2)*cos(q3)^2 + (4500767812266667*dq2*dq3*cos(q1)^2*cos(q2)^2*sin(q3))/16777216 + 321920000*dq2*dq4*cos(q2)^2*cos(q3)^2*sin(q1) + 482880000*d2q4*cos(q1)^2*cos(q2)*cos(q3)*sin(q3) + (4500767812266667*d2q3*cos(q1)^2*cos(q2)*sin(q2)*sin(q3))/33554432 + 160960000*d2q4*cos(q2)*cos(q3)^2*sin(q1)*sin(q2) + (4500767812266667*dq2^2*cos(q1)*sin(q1)*sin(q2)*sin(q3))/33554432 - (4500767812266667*dq3^2*cos(q1)*sin(q1)*sin(q2)*sin(q3))/33554432 - (4500767812266667*dq1*dq2*cos(q1)*cos(q3)*sin(q1))/16777216 - 160960000*dq1*dq3*cos(q2)*cos(q3)*sin(q1) - 160960000*dq1*dq4*cos(q1)*cos(q2)*sin(q2) + (4500767812266667*dq3*dq4*cos(q1)*cos(q2)*sin(q1))/16777216 + (4500767812266667*dq1*dq4*cos(q2)*cos(q3)*sin(q3))/16777216 + 482880000*dq1*dq4*cos(q1)^2*cos(q2)^2*cos(q3)^2 + (d2q1*l4^2*m4*sin(q2)*sin(q3))/8 - 482880000*dq2*dq3*cos(q1)*sin(q1)*sin(q3) - 241440000*dq1*dq3*cos(q2)*sin(q2)*sin(q3) + 241440000*dq2*dq4*cos(q3)*sin(q2)*sin(q3) + (d2q2*l2*l4*m4*cos(q4))/4 + 241440000*d2q4*cos(q1)*cos(q2)^2*cos(q3)^2*sin(q1) + (4500767812266667*dq3^2*cos(q1)^2*cos(q2)*cos(q3)*sin(q2))/33554432 - (4500767812266667*d2q4*cos(q1)*cos(q2)*cos(q3)*sin(q1)*sin(q3))/16777216 + 241440000*d2q3*cos(q1)*cos(q2)*sin(q1)*sin(q2)*sin(q3) + (dq1*dq2*l4^2*m4*cos(q2)*sin(q3))/4 + (dq1^2*l1*l4*m4*cos(q4)*sin(q2))/4 + (dq2^2*l2*l4*m4*cos(q3)*sin(q4))/4 - (g*l4*m4*cos(q4)*sin(q1)*sin(q2))/2 - (g*l4*m4*cos(q1)*sin(q3)*sin(q4))/2 + (dq1^2*l4^2*m4*cos(q2)^2*cos(q4)*sin(q4))/8 - (dq1^2*l4^2*m4*cos(q3)^2*cos(q4)*sin(q4))/8 + (dq2^2*l4^2*m4*cos(q3)^2*cos(q4)*sin(q4))/8 - (4500767812266667*dq1*dq4*cos(q1)*cos(q2)^2*cos(q3)^2*sin(q1))/16777216 - (4500767812266667*dq2*dq4*cos(q1)^2*cos(q2)*cos(q3)^2*sin(q2))/16777216 - (4500767812266667*dq3*dq4*cos(q1)^2*cos(q2)^2*cos(q3)*sin(q3))/16777216 + 241440000*dq3^2*cos(q1)*cos(q2)*cos(q3)*sin(q1)*sin(q2) - (dq2*dq3*l4^2*m4*cos(q4)^2*sin(q3))/4 - (dq1^2*l3*l4*m4*cos(q3)^2*sin(q4))/4 + (dq2^2*l3*l4*m4*cos(q3)^2*sin(q4))/4 + 160960000*dq2*dq4*cos(q1)*cos(q2)*cos(q3)*sin(q3) - 482880000*dq1*dq2*cos(q1)*cos(q2)*sin(q1)*sin(q3) + 482880000*dq1*dq3*cos(q1)*cos(q3)*sin(q1)*sin(q2) + 482880000*dq2*dq4*cos(q1)*cos(q2)*sin(q1)*sin(q2) - 482880000*dq3*dq4*cos(q1)*cos(q3)*sin(q1)*sin(q3) + 321920000*dq2*dq3*cos(q2)*sin(q1)*sin(q2)*sin(q3) - 160960000*dq1*dq4*cos(q3)*sin(q1)*sin(q2)*sin(q3) + (d2q2*l3*l4*m4*cos(q3)*cos(q4))/4 - (d2q1*l1*l4*m4*sin(q3)*sin(q4))/4 - (dq1^2*l4^2*m4*cos(q2)*cos(q3)*sin(q2))/8 + 160960000*dq1*dq4*cos(q1)*cos(q2)*cos(q3)^2*sin(q2) - (4500767812266667*dq1*dq4*cos(q1)^2*cos(q2)*cos(q3)*sin(q3))/8388608 - (4500767812266667*dq3*dq4*cos(q1)*cos(q2)*cos(q3)^2*sin(q1))/8388608 + 482880000*dq1*dq3*cos(q1)^2*cos(q2)*sin(q2)*sin(q3) + 482880000*dq2*dq3*cos(q1)*cos(q2)^2*sin(q1)*sin(q3) - 482880000*dq2*dq4*cos(q1)^2*cos(q3)*sin(q2)*sin(q3) - (g*l4*m4*cos(q2)*cos(q3)*sin(q1)*sin(q4))/2 + (dq1^2*l4^2*m4*cos(q2)*cos(q3)*cos(q4)^2*sin(q2))/4 + (dq1*dq3*l3*l4*m4*cos(q2)*sin(q4))/2 - (dq2*dq3*l3*l4*m4*cos(q4)*sin(q3))/2 - (dq1*dq2*l4^2*m4*cos(q2)*cos(q4)^2*sin(q3))/4 + (dq1*dq3*l4^2*m4*cos(q3)*cos(q4)^2*sin(q2))/4 + (dq1^2*l2*l4*m4*cos(q2)^2*cos(q3)*sin(q4))/4 - 965760000*dq1*dq4*cos(q1)*cos(q2)*cos(q3)*sin(q1)*sin(q3) + (dq1^2*l4^2*m4*cos(q2)^2*cos(q3)^2*cos(q4)*sin(q4))/8 - (4500767812266667*dq1*dq3*cos(q1)*cos(q2)*sin(q1)*sin(q2)*sin(q3))/16777216 + (4500767812266667*dq2*dq4*cos(q1)*cos(q3)*sin(q1)*sin(q2)*sin(q3))/16777216 - 321920000*dq3*dq4*cos(q2)*cos(q3)*sin(q1)*sin(q2)*sin(q3) - (d2q1*l2*l4*m4*cos(q2)*sin(q3)*sin(q4))/4 + (d2q1*l3*l4*m4*cos(q4)*sin(q2)*sin(q3))/4 + (dq1^2*l3*l4*m4*cos(q2)^2*cos(q3)^2*sin(q4))/4 - 482880000*dq2*dq4*cos(q1)*cos(q2)*cos(q3)^2*sin(q1)*sin(q2) - 482880000*dq3*dq4*cos(q1)*cos(q2)^2*cos(q3)*sin(q1)*sin(q3) + (dq1*dq3*l4^2*m4*cos(q2)*cos(q4)*sin(q4))/4 + (dq1^2*l1*l4*m4*cos(q2)*cos(q3)*sin(q4))/4 + (dq1^2*l2*l4*m4*cos(q2)*cos(q4)*sin(q2))/4 + (dq1*dq2*l2*l4*m4*sin(q2)*sin(q3)*sin(q4))/2 + (dq1^2*l3*l4*m4*cos(q2)*cos(q3)*cos(q4)*sin(q2))/4 + (dq1*dq3*l3*l4*m4*cos(q3)*cos(q4)*sin(q2))/2 + (dq1*dq2*l4^2*m4*cos(q3)*cos(q4)*sin(q2)*sin(q3)*sin(q4))/4 + (dq1*dq2*l3*l4*m4*cos(q3)*sin(q2)*sin(q3)*sin(q4))/2;
tao1= (90636232331764515*d2q1)/36893488147419103232 - (37193063271176147*dq2^2*cos(q1)^2)/36893488147419103232 + (14105118388521271*dq3^2*cos(q1)^2)/36893488147419103232 + (14105118388521271*dq3^2*cos(q2)^2)/73786976294838206464 - (8907563778312867*dq4^2*cos(q2)^2)/73786976294838206464 + (8907563778312867*dq4^2*cos(q3)^2)/73786976294838206464 + (58563985215450139*dq2^2*sin(2*q1))/73786976294838206464 - (1237161635876787*dq3^2*sin(2*q1))/18446744073709551616 + (17292715764458283*d2q2*cos(q1))/73786976294838206464 + (19796553826729791*d2q3*cos(q2))/36893488147419103232 + (37193063271176147*dq2^2)/73786976294838206464 - (14105118388521271*dq3^2)/73786976294838206464 - (14847907283222643*dq2*dq3*sin(q2))/36893488147419103232 + (5938375852208579*d2q4*cos(q1)*cos(q3))/73786976294838206464 - (14105118388521271*dq3^2*cos(q1)^2*cos(q2)^2)/36893488147419103232 + (8907563778312867*dq4^2*cos(q1)^2*cos(q2)^2)/36893488147419103232 - (8907563778312867*dq4^2*cos(q1)^2*cos(q3)^2)/36893488147419103232 + (8907563778312867*dq4^2*cos(q2)^2*cos(q3)^2)/73786976294838206464 + (11135930462416983*d2q3*sin(q1)*sin(q2))/73786976294838206464 + (6433240506559293*d2q4*sin(q2)*sin(q3))/18446744073709551616 + d2q1*l1^2*m1 + (d2q1*l1^2*m2)/2 + (d2q1*l1^2*m3)/2 + (d2q1*l1^2*m4)/2 + (d2q1*l3^2*m3)/8 + (d2q1*l3^2*m4)/2 + (d2q1*l4^2*m4)/8 + (8907563778312867*dq2*dq4*cos(q3))/36893488147419103232 + (1237161635876787*dq3^2*cos(q1)*cos(q2)^2*sin(q1))/9223372036854775808 - (1237161635876787*dq4^2*cos(q1)*cos(q2)^2*sin(q1))/9223372036854775808 + (1237161635876787*dq4^2*cos(q1)*cos(q3)^2*sin(q1))/9223372036854775808 + (d2q1*l2^2*m2*cos(q2)^2)/8 + (d2q1*l2^2*m3*cos(q2)^2)/2 + (d2q1*l2^2*m4*cos(q2)^2)/2 - (d2q1*l3^2*m3*cos(q3)^2)/8 - (d2q1*l3^2*m4*cos(q3)^2)/2 - (d2q1*l4^2*m4*cos(q2)^2)/8 - (8907563778312867*dq2*dq4*cos(q1)^2*cos(q3))/18446744073709551616 - (1237161635876787*dq2*dq3*cos(q1)^2*sin(q2))/4611686018427387904 - (5938375852208579*d2q4*cos(q2)*sin(q1)*sin(q3))/73786976294838206464 - (g*l1*m1*cos(q1))/2 - g*l1*m2*cos(q1) - g*l1*m3*cos(q1) - g*l1*m4*cos(q1) - (11135930462416983*dq3^2*cos(q1)*cos(q2)*sin(q2))/73786976294838206464 + (5938375852208579*dq4^2*cos(q1)*cos(q2)*sin(q2))/73786976294838206464 - (1237161635876787*dq4^2*cos(q2)*cos(q3)*sin(q3))/9223372036854775808 - (8907563778312867*dq4^2*cos(q1)^2*cos(q2)^2*cos(q3)^2)/36893488147419103232 + (d2q3*l3^2*m3*cos(q2))/8 + (d2q3*l3^2*m4*cos(q2))/2 + (11135930462416983*dq2*dq3*cos(q2)*sin(q1))/36893488147419103232 + (3958917234805719*dq2*dq4*cos(q2)*sin(q3))/18446744073709551616 - (5938375852208579*dq3*dq4*cos(q1)*sin(q3))/36893488147419103232 + (8907563778312867*dq3*dq4*cos(q3)*sin(q2))/18446744073709551616 + (d2q3*l4^2*m4*cos(q2)*cos(q4)^2)/8 + (1237161635876787*dq2*dq4*cos(q1)^2*cos(q2)*sin(q3))/4611686018427387904 + (5938375852208579*dq3*dq4*cos(q1)*cos(q2)^2*sin(q3))/36893488147419103232 - (1237161635876787*dq3*dq4*cos(q1)^2*cos(q3)*sin(q2))/4611686018427387904 + (1237161635876787*dq4^2*cos(q1)*cos(q2)^2*cos(q3)^2*sin(q1))/9223372036854775808 - (dq2*dq3*l3^2*m3*sin(q2))/4 - dq2*dq3*l3^2*m4*sin(q2) - (g*l2*m2*cos(q1)*cos(q2))/2 - g*l2*m3*cos(q1)*cos(q2) - g*l2*m4*cos(q1)*cos(q2) - (dq3^2*l1*l3*m3*sin(q3))/4 - (dq3^2*l1*l3*m4*sin(q3))/2 + (d2q1*l3^2*m3*cos(q2)^2*cos(q3)^2)/8 + (d2q1*l3^2*m4*cos(q2)^2*cos(q3)^2)/2 + (d2q1*l4^2*m4*cos(q2)^2*cos(q4)^2)/8 - (d2q1*l4^2*m4*cos(q3)^2*cos(q4)^2)/8 + (g*l3*m3*sin(q1)*sin(q3))/2 + g*l3*m4*sin(q1)*sin(q3) - (dq1*dq2*l2^2*m2*sin(2*q2))/8 - (dq1*dq2*l2^2*m3*sin(2*q2))/2 - (dq1*dq2*l2^2*m4*sin(2*q2))/2 + (dq1*dq2*l4^2*m4*sin(2*q2))/8 + (dq1*dq3*l3^2*m3*sin(2*q3))/8 + (dq1*dq3*l3^2*m4*sin(2*q3))/2 + (5938375852208579*dq4^2*cos(q3)*sin(q1)*sin(q2)*sin(q3))/73786976294838206464 + (1237161635876787*dq2*dq4*cos(q1)*cos(q3)*sin(q1))/4611686018427387904 + (d2q4*l4^2*m4*sin(q2)*sin(q3))/8 - (14105118388521271*dq2*dq3*cos(q1)*sin(q1)*sin(q2))/18446744073709551616 + (8907563778312867*dq3*dq4*cos(q2)*sin(q2)*sin(q3))/36893488147419103232 + (5938375852208579*dq2*dq4*sin(q1)*sin(q2)*sin(q3))/36893488147419103232 + (d2q1*l1*l2*m2*cos(q2))/2 + d2q1*l1*l2*m3*cos(q2) + d2q1*l1*l2*m4*cos(q2) + (d2q3*l1*l3*m3*cos(q3))/4 + (d2q3*l1*l3*m4*cos(q3))/2 + (d2q1*l3*l4*m4*cos(q4))/2 - (5938375852208579*dq4^2*cos(q1)*cos(q2)*cos(q3)^2*sin(q2))/73786976294838206464 + (1237161635876787*dq4^2*cos(q1)^2*cos(q2)*cos(q3)*sin(q3))/4611686018427387904 + (d2q1*l2*l3*m3*cos(q2)^2*cos(q3))/2 + d2q1*l2*l3*m4*cos(q2)^2*cos(q3) - (d2q1*l3*l4*m4*cos(q3)^2*cos(q4))/2 + (dq3*dq4*l4^2*m4*cos(q3)*sin(q2))/4 - (g*l3*m3*cos(q1)*cos(q2)*cos(q3))/2 - g*l3*m4*cos(q1)*cos(q2)*cos(q3) + (dq2^2*l2*l3*m3*cos(q2)*sin(q3))/4 + (dq2^2*l2*l3*m4*cos(q2)*sin(q3))/2 - (dq3^2*l2*l3*m3*cos(q2)*sin(q3))/4 - (dq3^2*l2*l3*m4*cos(q2)*sin(q3))/2 - (dq3^2*l1*l4*m4*cos(q4)*sin(q3))/4 - (dq4^2*l1*l4*m4*cos(q4)*sin(q3))/4 + (g*l4*m4*cos(q1)*sin(q2)*sin(q4))/2 + (g*l4*m4*cos(q4)*sin(q1)*sin(q3))/2 - (dq1*dq2*l1*l2*m2*sin(q2))/2 - dq1*dq2*l1*l2*m3*sin(q2) - dq1*dq2*l1*l2*m4*sin(q2) + (dq1*dq2*l2*l4*m4*sin(q4))/2 - (dq1*dq4*l3*l4*m4*sin(q4))/2 + (8907563778312867*dq4^2*cos(q1)*cos(q2)*cos(q3)*sin(q1)*sin(q3))/18446744073709551616 + (dq2*dq3*l3^2*m3*cos(q3)^2*sin(q2))/4 + dq2*dq3*l3^2*m4*cos(q3)^2*sin(q2) - (dq2*dq3*l4^2*m4*cos(q4)^2*sin(q2))/4 + (d2q1*l4^2*m4*cos(q2)^2*cos(q3)^2*cos(q4)^2)/8 + (d2q2*l3^2*m3*cos(q3)*sin(q2)*sin(q3))/8 + (d2q2*l3^2*m4*cos(q3)*sin(q2)*sin(q3))/2 + (8907563778312867*dq2*dq4*cos(q1)*cos(q2)*sin(q1)*sin(q3))/18446744073709551616 - (8907563778312867*dq3*dq4*cos(q1)*cos(q3)*sin(q1)*sin(q2))/18446744073709551616 + (d2q1*l1*l3*m3*cos(q2)*cos(q3))/2 + d2q1*l1*l3*m4*cos(q2)*cos(q3) + (d2q3*l2*l3*m3*cos(q2)*cos(q3))/4 + (d2q3*l2*l3*m4*cos(q2)*cos(q3))/2 + (d2q3*l1*l4*m4*cos(q3)*cos(q4))/4 + (d2q3*l3*l4*m4*cos(q2)*cos(q4))/2 + (d2q2*l2*l3*m3*sin(q2)*sin(q3))/4 - (d2q1*l1*l4*m4*sin(q2)*sin(q4))/2 + (d2q2*l2*l3*m4*sin(q2)*sin(q3))/2 - (d2q4*l1*l4*m4*sin(q3)*sin(q4))/4 + (dq2^2*l3^2*m3*cos(q2)*cos(q3)*sin(q3))/8 + (dq2^2*l3^2*m4*cos(q2)*cos(q3)*sin(q3))/2 - (8907563778312867*dq3*dq4*cos(q1)^2*cos(q2)*sin(q2)*sin(q3))/18446744073709551616 - (dq2^2*l3*l4*m4*sin(q2)*sin(q3)*sin(q4))/4 + (dq3^2*l3*l4*m4*sin(q2)*sin(q3)*sin(q4))/4 - (dq4^2*l3*l4*m4*sin(q2)*sin(q3)*sin(q4))/4 + (dq2^2*l4^2*m4*cos(q2)*cos(q3)*cos(q4)^2*sin(q3))/8 - (dq1*dq2*l1*l3*m3*cos(q3)*sin(q2))/2 - dq1*dq2*l1*l3*m4*cos(q3)*sin(q2) - (dq1*dq3*l1*l3*m3*cos(q2)*sin(q3))/2 - dq1*dq3*l1*l3*m4*cos(q2)*sin(q3) - (dq1*dq2*l1*l4*m4*cos(q2)*sin(q4))/2 - (dq1*dq4*l1*l4*m4*cos(q4)*sin(q2))/2 + (dq1*dq2*l3*l4*m4*cos(q3)*sin(q4))/2 - dq2*dq3*l3*l4*m4*cos(q4)*sin(q2) - (dq3*dq4*l1*l4*m4*cos(q3)*sin(q4))/2 - (dq3*dq4*l3*l4*m4*cos(q2)*sin(q4))/2 + (d2q1*l3*l4*m4*cos(q2)^2*cos(q3)^2*cos(q4))/2 - (dq1*dq2*l3^2*m3*cos(q2)*cos(q3)^2*sin(q2))/4 - dq1*dq2*l3^2*m4*cos(q2)*cos(q3)^2*sin(q2) - (dq1*dq3*l3^2*m3*cos(q2)^2*cos(q3)*sin(q3))/4 - (dq1*dq2*l4^2*m4*cos(q2)*cos(q4)^2*sin(q2))/4 - dq1*dq3*l3^2*m4*cos(q2)^2*cos(q3)*sin(q3) + (dq1*dq3*l4^2*m4*cos(q3)*cos(q4)^2*sin(q3))/4 - (dq1*dq4*l4^2*m4*cos(q2)^2*cos(q4)*sin(q4))/4 + (dq2*dq4*l4^2*m4*cos(q2)*cos(q4)^2*sin(q3))/4 + (dq1*dq4*l4^2*m4*cos(q3)^2*cos(q4)*sin(q4))/4 - (dq3*dq4*l4^2*m4*cos(q3)*cos(q4)^2*sin(q2))/4 + (d2q2*l4^2*m4*cos(q2)*cos(q4)*sin(q3)*sin(q4))/8 - (d2q3*l4^2*m4*cos(q3)*cos(q4)*sin(q2)*sin(q4))/8 + (1237161635876787*dq3*dq4*cos(q1)*cos(q2)*sin(q1)*sin(q2)*sin(q3))/4611686018427387904 - (dq1*dq3*l2*l3*m3*cos(q2)^2*sin(q3))/2 - dq1*dq3*l2*l3*m4*cos(q2)^2*sin(q3) - dq1*dq2*l2*l4*m4*cos(q2)^2*sin(q4) + (dq1*dq4*l3*l4*m4*cos(q3)^2*sin(q4))/2 + (d2q1*l1*l4*m4*cos(q2)*cos(q3)*cos(q4))/2 + (d2q3*l2*l4*m4*cos(q2)*cos(q3)*cos(q4))/4 - (d2q1*l2*l4*m4*cos(q2)*sin(q2)*sin(q4))/2 + (d2q2*l2*l4*m4*cos(q4)*sin(q2)*sin(q3))/4 + (d2q2*l3*l4*m4*cos(q2)*sin(q3)*sin(q4))/4 - (d2q3*l3*l4*m4*cos(q3)*sin(q2)*sin(q4))/4 - (d2q4*l2*l4*m4*cos(q2)*sin(q3)*sin(q4))/4 + (d2q4*l3*l4*m4*cos(q4)*sin(q2)*sin(q3))/4 + (dq2*dq3*l4^2*m4*cos(q3)^2*cos(q4)^2*sin(q2))/4 + (d2q2*l4^2*m4*cos(q3)*cos(q4)^2*sin(q2)*sin(q3))/8 - (dq2^2*l4^2*m4*cos(q4)*sin(q2)*sin(q3)*sin(q4))/8 + (dq3^2*l4^2*m4*cos(q4)*sin(q2)*sin(q3)*sin(q4))/8 + (d2q1*l2*l4*m4*cos(q2)^2*cos(q3)*cos(q4))/2 + (dq1*dq4*l4^2*m4*cos(q2)*cos(q3)*sin(q2))/4 + (dq1*dq2*l4^2*m4*cos(q3)*cos(q4)*sin(q4))/4 - (dq3*dq4*l4^2*m4*cos(q2)*cos(q4)*sin(q4))/4 - (g*l4*m4*cos(q1)*cos(q2)*cos(q3)*cos(q4))/2 + (dq2^2*l2*l4*m4*cos(q2)*cos(q4)*sin(q3))/4 - (dq3^2*l2*l4*m4*cos(q2)*cos(q4)*sin(q3))/4 - (dq4^2*l2*l4*m4*cos(q2)*cos(q4)*sin(q3))/4 - (dq1*dq2*l4^2*m4*cos(q2)^2*cos(q3)*cos(q4)*sin(q4))/2 - (dq1*dq4*l4^2*m4*cos(q2)*cos(q3)*cos(q4)^2*sin(q2))/2 - (d2q1*l4^2*m4*cos(q2)*cos(q3)*cos(q4)*sin(q2)*sin(q4))/4 - dq1*dq2*l3*l4*m4*cos(q2)^2*cos(q3)*sin(q4) - (dq1*dq3*l2*l4*m4*cos(q2)^2*cos(q4)*sin(q3))/2 - (dq1*dq4*l2*l4*m4*cos(q2)^2*cos(q3)*sin(q4))/2 + dq2*dq3*l3*l4*m4*cos(q3)^2*cos(q4)*sin(q2) - (d2q1*l3*l4*m4*cos(q2)*cos(q3)*sin(q2)*sin(q4))/2 + (d2q2*l3*l4*m4*cos(q3)*cos(q4)*sin(q2)*sin(q3))/2 - (dq1*dq2*l4^2*m4*cos(q2)*cos(q3)^2*cos(q4)^2*sin(q2))/4 - (dq1*dq3*l4^2*m4*cos(q2)^2*cos(q3)*cos(q4)^2*sin(q3))/4 - (dq1*dq4*l4^2*m4*cos(q2)^2*cos(q3)^2*cos(q4)*sin(q4))/4 - (dq1*dq4*l3*l4*m4*cos(q2)^2*cos(q3)^2*sin(q4))/2 + (dq2^2*l3*l4*m4*cos(q2)*cos(q3)*cos(q4)*sin(q3))/2 - dq1*dq2*l2*l3*m3*cos(q2)*cos(q3)*sin(q2) - 2*dq1*dq2*l2*l3*m4*cos(q2)*cos(q3)*sin(q2) - (dq1*dq2*l1*l4*m4*cos(q3)*cos(q4)*sin(q2))/2 - (dq1*dq3*l1*l4*m4*cos(q2)*cos(q4)*sin(q3))/2 - (dq1*dq4*l1*l4*m4*cos(q2)*cos(q3)*sin(q4))/2 - (dq1*dq4*l2*l4*m4*cos(q2)*cos(q4)*sin(q2))/2 + dq1*dq3*l3*l4*m4*cos(q3)*cos(q4)*sin(q3) + (dq2*dq4*l3*l4*m4*cos(q2)*cos(q4)*sin(q3))/2 - (dq3*dq4*l2*l4*m4*cos(q2)*cos(q3)*sin(q4))/2 - dq1*dq2*l3*l4*m4*cos(q2)*cos(q3)^2*cos(q4)*sin(q2) - dq1*dq3*l3*l4*m4*cos(q2)^2*cos(q3)*cos(q4)*sin(q3) + (dq1*dq3*l4^2*m4*cos(q2)*cos(q4)*sin(q2)*sin(q3)*sin(q4))/4 - (dq2*dq4*l4^2*m4*cos(q3)*cos(q4)*sin(q2)*sin(q3)*sin(q4))/4 - dq1*dq2*l2*l4*m4*cos(q2)*cos(q3)*cos(q4)*sin(q2) - (dq1*dq4*l3*l4*m4*cos(q2)*cos(q3)*cos(q4)*sin(q2))/2 + (dq1*dq3*l3*l4*m4*cos(q2)*sin(q2)*sin(q3)*sin(q4))/2 - (dq2*dq4*l3*l4*m4*cos(q3)*sin(q2)*sin(q3)*sin(q4))/2;
tao2= (5764238588152761*d2q2)/9223372036854775808 + (37193063271176147*d2q2*sin(2*q1))/73786976294838206464 - (17292715764458283*dq1^2*sin(q1))/73786976294838206464 + (11135930462416983*dq3^2*sin(q1))/73786976294838206464 - (5938375852208579*dq4^2*sin(q1))/73786976294838206464 - (37193063271176147*dq1*dq2)/36893488147419103232 + (17292715764458283*d2q1*cos(q1))/73786976294838206464 + (3958917234805719*d2q4*cos(q3))/18446744073709551616 + (14105118388521271*d2q3*sin(q2))/73786976294838206464 + (58563985215450139*d2q2*cos(q1)^2)/36893488147419103232 + (14847907283222643*dq1*dq3*sin(q2))/36893488147419103232 - (3958917234805719*dq3*dq4*sin(q3))/18446744073709551616 - (11135930462416983*dq3^2*cos(q2)^2*sin(q1))/36893488147419103232 + (5938375852208579*dq4^2*cos(q2)^2*sin(q1))/36893488147419103232 + (5938375852208579*dq4^2*cos(q3)^2*sin(q1))/73786976294838206464 + (37193063271176147*dq1*dq2*cos(q1)^2)/18446744073709551616 - (58563985215450139*dq1*dq2*sin(2*q1))/36893488147419103232 + (11135930462416983*d2q3*cos(q1)*cos(q2))/73786976294838206464 - (8907563778312867*d2q4*cos(q2)*sin(q3))/73786976294838206464 + (1237161635876787*d2q4*cos(q1)^2*cos(q3))/9223372036854775808 - (14105118388521271*d2q3*cos(q1)^2*sin(q2))/36893488147419103232 + (d2q2*l2^2*m2)/8 + (d2q2*l2^2*m3)/2 + (d2q2*l2^2*m4)/2 + (d2q2*l4^2*m4)/8 - (8907563778312867*dq1*dq4*cos(q3))/36893488147419103232 + (1237161635876787*dq3^2*cos(q1)^2*cos(q2)*sin(q2))/9223372036854775808 - (1237161635876787*dq4^2*cos(q1)^2*cos(q2)*sin(q2))/9223372036854775808 + (d2q2*l3^2*m3*cos(q3)^2)/8 + (d2q2*l3^2*m4*cos(q3)^2)/2 - (d2q2*l4^2*m4*cos(q4)^2)/8 + (8907563778312867*dq1*dq4*cos(q1)^2*cos(q3))/18446744073709551616 + (1237161635876787*dq1*dq3*cos(q1)^2*sin(q2))/4611686018427387904 + (8907563778312867*d2q4*cos(q1)*cos(q3)*sin(q1))/36893488147419103232 + (1237161635876787*d2q3*cos(q1)*sin(q1)*sin(q2))/9223372036854775808 + (5938375852208579*d2q4*cos(q1)*sin(q2)*sin(q3))/73786976294838206464 - (5938375852208579*dq4^2*cos(q2)^2*cos(q3)^2*sin(q1))/36893488147419103232 + (dq1^2*l2^2*m2*sin(2*q2))/16 + (dq1^2*l2^2*m3*sin(2*q2))/4 + (dq1^2*l2^2*m4*sin(2*q2))/4 - (dq1^2*l4^2*m4*sin(2*q2))/16 + (8907563778312867*d2q4*cos(q1)^2*cos(q2)*sin(q3))/36893488147419103232 - (8907563778312867*dq4^2*cos(q3)*sin(q2)*sin(q3))/73786976294838206464 + (d2q4*l4^2*m4*cos(q3))/8 - (8907563778312867*dq3*dq4*cos(q2)*cos(q3))/36893488147419103232 - (11135930462416983*dq1*dq3*cos(q2)*sin(q1))/36893488147419103232 - (3958917234805719*dq1*dq4*cos(q2)*sin(q3))/18446744073709551616 + (8907563778312867*dq3*dq4*cos(q1)^2*cos(q2)*cos(q3))/18446744073709551616 - (1237161635876787*dq1*dq4*cos(q1)^2*cos(q2)*sin(q3))/4611686018427387904 - (1237161635876787*d2q4*cos(q1)*cos(q2)*sin(q1)*sin(q3))/9223372036854775808 + (1237161635876787*dq4^2*cos(q1)^2*cos(q2)*cos(q3)^2*sin(q2))/9223372036854775808 - (dq3*dq4*l4^2*m4*sin(q3))/4 + (dq1^2*l1*l2*m2*sin(q2))/4 + (dq1^2*l1*l2*m3*sin(q2))/2 + (dq1^2*l1*l2*m4*sin(q2))/2 - (dq1^2*l2*l4*m4*sin(q4))/4 - (dq4^2*l2*l4*m4*sin(q4))/4 + (d2q2*l4^2*m4*cos(q3)^2*cos(q4)^2)/8 + (g*l2*m2*sin(q1)*sin(q2))/2 + g*l2*m3*sin(q1)*sin(q2) + g*l2*m4*sin(q1)*sin(q2) - (1237161635876787*dq3*dq4*cos(q1)^2*cos(q2)^2*sin(q3))/4611686018427387904 - (5938375852208579*dq4^2*cos(q1)*cos(q2)*cos(q3)*sin(q3))/73786976294838206464 + (14105118388521271*dq3^2*cos(q1)*cos(q2)*sin(q1)*sin(q2))/36893488147419103232 - (8907563778312867*dq4^2*cos(q1)*cos(q2)*sin(q1)*sin(q2))/36893488147419103232 - (dq2*dq3*l3^2*m3*sin(2*q3))/8 - (dq2*dq3*l3^2*m4*sin(2*q3))/2 + (dq2*dq4*l4^2*m4*sin(2*q4))/8 - (1237161635876787*dq1*dq4*cos(q1)*cos(q3)*sin(q1))/4611686018427387904 + (5938375852208579*dq3*dq4*cos(q1)*cos(q3)*sin(q2))/36893488147419103232 + (14105118388521271*dq1*dq3*cos(q1)*sin(q1)*sin(q2))/18446744073709551616 - (5938375852208579*dq1*dq4*sin(q1)*sin(q2)*sin(q3))/36893488147419103232 + (d2q2*l2*l3*m3*cos(q3))/2 + d2q2*l2*l3*m4*cos(q3) + (d2q4*l2*l4*m4*cos(q4))/4 + (8907563778312867*dq4^2*cos(q1)^2*cos(q3)*sin(q2)*sin(q3))/36893488147419103232 + (d2q2*l3*l4*m4*cos(q3)^2*cos(q4))/2 - (dq1*dq4*l4^2*m4*cos(q2)*sin(q3))/4 + (dq1^2*l1*l3*m3*cos(q3)*sin(q2))/4 + (dq1^2*l1*l3*m4*cos(q3)*sin(q2))/2 + (dq1^2*l1*l4*m4*cos(q2)*sin(q4))/4 - (dq1^2*l3*l4*m4*cos(q3)*sin(q4))/4 + (dq3^2*l3*l4*m4*cos(q3)*sin(q4))/4 - (dq4^2*l3*l4*m4*cos(q3)*sin(q4))/4 + (g*l3*m3*cos(q3)*sin(q1)*sin(q2))/2 + g*l3*m4*cos(q3)*sin(q1)*sin(q2) + (g*l4*m4*cos(q2)*sin(q1)*sin(q4))/2 + (dq1^2*l3^2*m3*cos(q2)*cos(q3)^2*sin(q2))/8 + (dq1^2*l3^2*m4*cos(q2)*cos(q3)^2*sin(q2))/2 + (dq1^2*l4^2*m4*cos(q2)*cos(q4)^2*sin(q2))/8 - (dq2*dq3*l2*l3*m3*sin(q3))/2 - dq2*dq3*l2*l3*m4*sin(q3) + (dq1*dq3*l3^2*m3*cos(q3)^2*sin(q2))/4 + dq1*dq3*l3^2*m4*cos(q3)^2*sin(q2) + (dq3*dq4*l4^2*m4*cos(q4)^2*sin(q3))/4 - (1237161635876787*dq4^2*cos(q1)*cos(q3)*sin(q1)*sin(q2)*sin(q3))/9223372036854775808 + (dq1^2*l2*l4*m4*cos(q2)^2*sin(q4))/2 - (1237161635876787*dq3*dq4*cos(q1)*cos(q2)*cos(q3)*sin(q1))/4611686018427387904 + (d2q1*l3^2*m3*cos(q3)*sin(q2)*sin(q3))/8 + (d2q1*l3^2*m4*cos(q3)*sin(q2)*sin(q3))/2 + (d2q3*l4^2*m4*cos(q4)*sin(q3)*sin(q4))/8 - (8907563778312867*dq1*dq4*cos(q1)*cos(q2)*sin(q1)*sin(q3))/18446744073709551616 - (5938375852208579*dq3*dq4*cos(q2)*sin(q1)*sin(q2)*sin(q3))/18446744073709551616 + (d2q2*l2*l4*m4*cos(q3)*cos(q4))/2 + (d2q4*l3*l4*m4*cos(q3)*cos(q4))/4 + (8907563778312867*dq4^2*cos(q1)*cos(q2)*cos(q3)^2*sin(q1)*sin(q2))/36893488147419103232 + (d2q1*l2*l3*m3*sin(q2)*sin(q3))/4 + (d2q1*l2*l3*m4*sin(q2)*sin(q3))/2 + (d2q3*l3*l4*m4*sin(q3)*sin(q4))/4 - (dq1^2*l4^2*m4*cos(q3)*cos(q4)*sin(q4))/8 + (dq3^2*l4^2*m4*cos(q3)*cos(q4)*sin(q4))/8 - (8907563778312867*dq3*dq4*cos(q1)*cos(q2)^2*sin(q1)*sin(q3))/18446744073709551616 + (g*l4*m4*cos(q3)*cos(q4)*sin(q1)*sin(q2))/2 + (dq1^2*l4^2*m4*cos(q2)^2*cos(q3)*cos(q4)*sin(q4))/4 + (dq1*dq3*l2*l3*m3*cos(q3)*sin(q2))/2 + dq1*dq3*l2*l3*m4*cos(q3)*sin(q2) - (dq2*dq3*l2*l4*m4*cos(q4)*sin(q3))/2 - (dq2*dq4*l2*l4*m4*cos(q3)*sin(q4))/2 + (dq1*dq4*l4^2*m4*cos(q2)*cos(q4)^2*sin(q3))/4 - (dq2*dq3*l4^2*m4*cos(q3)*cos(q4)^2*sin(q3))/4 - (dq2*dq4*l4^2*m4*cos(q3)^2*cos(q4)*sin(q4))/4 + (dq1^2*l3*l4*m4*cos(q2)^2*cos(q3)*sin(q4))/2 + (d2q1*l4^2*m4*cos(q2)*cos(q4)*sin(q3)*sin(q4))/8 + (dq1^2*l4^2*m4*cos(q2)*cos(q3)^2*cos(q4)^2*sin(q2))/8 - (dq2*dq4*l3*l4*m4*cos(q3)^2*sin(q4))/2 + (d2q1*l2*l4*m4*cos(q4)*sin(q2)*sin(q3))/4 + (d2q1*l3*l4*m4*cos(q2)*sin(q3)*sin(q4))/4 + (dq1*dq3*l4^2*m4*cos(q3)^2*cos(q4)^2*sin(q2))/4 + (d2q1*l4^2*m4*cos(q3)*cos(q4)^2*sin(q2)*sin(q3))/8 + (dq1^2*l2*l3*m3*cos(q2)*cos(q3)*sin(q2))/2 + dq1^2*l2*l3*m4*cos(q2)*cos(q3)*sin(q2) + (dq1^2*l1*l4*m4*cos(q3)*cos(q4)*sin(q2))/4 - (dq1*dq4*l2*l4*m4*sin(q2)*sin(q3)*sin(q4))/2 + (dq1^2*l3*l4*m4*cos(q2)*cos(q3)^2*cos(q4)*sin(q2))/2 + dq1*dq3*l3*l4*m4*cos(q3)^2*cos(q4)*sin(q2) + (d2q1*l3*l4*m4*cos(q3)*cos(q4)*sin(q2)*sin(q3))/2 + (dq1*dq3*l4^2*m4*cos(q2)*cos(q3)*cos(q4)*sin(q4))/4 + (dq1^2*l2*l4*m4*cos(q2)*cos(q3)*cos(q4)*sin(q2))/2 + (dq1*dq3*l2*l4*m4*cos(q3)*cos(q4)*sin(q2))/2 + (dq1*dq3*l3*l4*m4*cos(q2)*cos(q3)*sin(q4))/2 - dq2*dq3*l3*l4*m4*cos(q3)*cos(q4)*sin(q3) - (dq1*dq4*l4^2*m4*cos(q3)*cos(q4)*sin(q2)*sin(q3)*sin(q4))/4 - (dq1*dq4*l3*l4*m4*cos(q3)*sin(q2)*sin(q3)*sin(q4))/2;
tao3= (19796553826729791*d2q3)/36893488147419103232 - (14105118388521271*d2q3*sin(2*q1))/73786976294838206464 + (14105118388521271*dq1*dq3)/36893488147419103232 - (1237161635876787*dq4^2*sin(2*q3))/18446744073709551616 + (19796553826729791*d2q1*cos(q2))/36893488147419103232 + (14105118388521271*d2q2*sin(q2))/73786976294838206464 - (1237161635876787*d2q3*cos(q1)^2)/9223372036854775808 + (14105118388521271*dq2^2*cos(q2))/73786976294838206464 - (8907563778312867*dq4^2*cos(q2))/73786976294838206464 - (24745200370236939*dq1*dq2*sin(q2))/36893488147419103232 - (11135930462416983*dq2*dq3*sin(q1))/36893488147419103232 + (3958917234805719*dq2*dq4*sin(q3))/18446744073709551616 + (1237161635876787*d2q3*cos(q1)^2*cos(q2)^2)/9223372036854775808 - (14105118388521271*dq2^2*cos(q1)^2*cos(q2))/36893488147419103232 + (8907563778312867*dq4^2*cos(q1)^2*cos(q2))/36893488147419103232 + (8907563778312867*dq4^2*cos(q2)*cos(q3)^2)/36893488147419103232 - (14105118388521271*dq1*dq3*cos(q1)^2)/18446744073709551616 - (14105118388521271*dq1*dq3*cos(q2)^2)/36893488147419103232 + (1237161635876787*dq1*dq3*sin(2*q1))/9223372036854775808 + (11135930462416983*d2q2*cos(q1)*cos(q2))/73786976294838206464 + (8907563778312867*d2q4*cos(q3)*sin(q2))/73786976294838206464 + (11135930462416983*d2q1*sin(q1)*sin(q2))/73786976294838206464 + (5938375852208579*d2q4*sin(q1)*sin(q3))/73786976294838206464 - (14105118388521271*d2q2*cos(q1)^2*sin(q2))/36893488147419103232 + (11135930462416983*dq1^2*cos(q1)*sin(q2))/73786976294838206464 - (11135930462416983*dq2^2*cos(q1)*sin(q2))/73786976294838206464 + (5938375852208579*dq4^2*cos(q1)*sin(q2))/73786976294838206464 + (d2q3*l3^2*m3)/8 + (d2q3*l3^2*m4)/2 - (5938375852208579*dq4^2*cos(q1)*cos(q3)^2*sin(q2))/36893488147419103232 + (1237161635876787*dq4^2*cos(q1)^2*cos(q3)*sin(q3))/9223372036854775808 + (d2q3*l4^2*m4*cos(q4)^2)/8 + (1237161635876787*dq1*dq2*cos(q1)^2*sin(q2))/4611686018427387904 + (11135930462416983*dq2*dq3*cos(q2)^2*sin(q1))/18446744073709551616 + (5938375852208579*d2q4*cos(q1)*cos(q2)*cos(q3))/73786976294838206464 - (8907563778312867*dq4^2*cos(q1)^2*cos(q2)*cos(q3)^2)/18446744073709551616 + (1237161635876787*d2q2*cos(q1)*sin(q1)*sin(q2))/9223372036854775808 + (11135930462416983*d2q3*cos(q2)*sin(q1)*sin(q2))/36893488147419103232 + (14105118388521271*dq1*dq3*cos(q1)^2*cos(q2)^2)/18446744073709551616 - (dq1^2*l3^2*m3*sin(2*q3))/16 - (dq1^2*l3^2*m4*sin(2*q3))/4 + (dq2^2*l3^2*m3*sin(2*q3))/16 + (dq2^2*l3^2*m4*sin(2*q3))/4 + (14105118388521271*d2q3*cos(q1)*cos(q2)^2*sin(q1))/36893488147419103232 - (8907563778312867*d2q4*cos(q1)^2*cos(q3)*sin(q2))/36893488147419103232 + (1237161635876787*dq2^2*cos(q1)*cos(q2)*sin(q1))/9223372036854775808 - (1237161635876787*dq4^2*cos(q1)*cos(q2)*sin(q1))/9223372036854775808 - (5938375852208579*d2q4*cos(q2)^2*sin(q1)*sin(q3))/36893488147419103232 + (d2q1*l3^2*m3*cos(q2))/8 + (d2q1*l3^2*m4*cos(q2))/2 + (8907563778312867*dq2*dq4*cos(q2)*cos(q3))/36893488147419103232 + (5938375852208579*dq1*dq4*cos(q1)*sin(q3))/36893488147419103232 - (8907563778312867*dq1*dq4*cos(q3)*sin(q2))/18446744073709551616 + (d2q1*l4^2*m4*cos(q2)*cos(q4)^2)/8 - (8907563778312867*dq2*dq4*cos(q1)^2*cos(q2)*cos(q3))/18446744073709551616 - (1237161635876787*dq1*dq3*cos(q1)*cos(q2)^2*sin(q1))/4611686018427387904 - (1237161635876787*dq2*dq3*cos(q1)^2*cos(q2)*sin(q2))/4611686018427387904 - (5938375852208579*dq1*dq4*cos(q1)*cos(q2)^2*sin(q3))/36893488147419103232 + (1237161635876787*dq1*dq4*cos(q1)^2*cos(q3)*sin(q2))/4611686018427387904 + (1237161635876787*d2q4*cos(q1)*cos(q3)*sin(q1)*sin(q2))/9223372036854775808 + (1237161635876787*dq4^2*cos(q1)^2*cos(q2)^2*cos(q3)*sin(q3))/9223372036854775808 - (g*l3*m3*cos(q1)*cos(q3))/2 - g*l3*m4*cos(q1)*cos(q3) + (dq2^2*l2*l3*m3*sin(q3))/4 + (dq2^2*l2*l3*m4*sin(q3))/2 + (1237161635876787*dq2*dq4*cos(q1)^2*cos(q2)^2*sin(q3))/4611686018427387904 + (1237161635876787*d2q4*cos(q1)^2*cos(q2)*sin(q2)*sin(q3))/9223372036854775808 + (8907563778312867*dq4^2*cos(q1)*cos(q3)*sin(q1)*sin(q3))/36893488147419103232 - (dq3*dq4*l4^2*m4*sin(2*q4))/8 + (11135930462416983*dq1*dq3*cos(q1)*cos(q2)*sin(q2))/36893488147419103232 - (5938375852208579*dq2*dq4*cos(q1)*cos(q3)*sin(q2))/36893488147419103232 + (14105118388521271*dq1*dq2*cos(q1)*sin(q1)*sin(q2))/18446744073709551616 - (8907563778312867*dq1*dq4*cos(q2)*sin(q2)*sin(q3))/36893488147419103232 + (d2q1*l1*l3*m3*cos(q3))/4 + (d2q1*l1*l3*m4*cos(q3))/2 + (d2q3*l3*l4*m4*cos(q4))/2 + (1237161635876787*dq4^2*cos(q1)*cos(q2)*cos(q3)^2*sin(q1))/4611686018427387904 + (8907563778312867*d2q4*cos(q1)*cos(q2)*sin(q1)*sin(q2)*sin(q3))/36893488147419103232 - (g*l4*m4*cos(q1)*cos(q3)*cos(q4))/2 + (dq1^2*l1*l3*m3*cos(q2)*sin(q3))/4 + (dq1^2*l1*l3*m4*cos(q2)*sin(q3))/2 + (dq2^2*l2*l4*m4*cos(q4)*sin(q3))/4 + (g*l3*m3*cos(q2)*sin(q1)*sin(q3))/2 + g*l3*m4*cos(q2)*sin(q1)*sin(q3) + (dq1^2*l3^2*m3*cos(q2)^2*cos(q3)*sin(q3))/8 + (dq1^2*l3^2*m4*cos(q2)^2*cos(q3)*sin(q3))/2 - (dq1^2*l4^2*m4*cos(q3)*cos(q4)^2*sin(q3))/8 + (dq2^2*l4^2*m4*cos(q3)*cos(q4)^2*sin(q3))/8 - (dq3*dq4*l3*l4*m4*sin(q4))/2 - (dq1*dq2*l3^2*m3*cos(q3)^2*sin(q2))/4 - dq1*dq2*l3^2*m4*cos(q3)^2*sin(q2) + (dq2*dq4*l4^2*m4*cos(q4)^2*sin(q3))/4 + (5938375852208579*dq4^2*cos(q2)*cos(q3)*sin(q1)*sin(q2)*sin(q3))/36893488147419103232 + (dq1^2*l2*l3*m3*cos(q2)^2*sin(q3))/4 + (dq1^2*l2*l3*m4*cos(q2)^2*sin(q3))/2 + (1237161635876787*dq2*dq4*cos(q1)*cos(q2)*cos(q3)*sin(q1))/4611686018427387904 + (d2q2*l4^2*m4*cos(q4)*sin(q3)*sin(q4))/8 - (14105118388521271*dq2*dq3*cos(q1)*cos(q2)*sin(q1)*sin(q2))/18446744073709551616 + (8907563778312867*dq1*dq4*cos(q1)*cos(q3)*sin(q1)*sin(q2))/18446744073709551616 + (5938375852208579*dq2*dq4*cos(q2)*sin(q1)*sin(q2)*sin(q3))/18446744073709551616 + (d2q1*l2*l3*m3*cos(q2)*cos(q3))/4 + (d2q1*l2*l3*m4*cos(q2)*cos(q3))/2 + (d2q1*l1*l4*m4*cos(q3)*cos(q4))/4 + (d2q1*l3*l4*m4*cos(q2)*cos(q4))/2 + (8907563778312867*dq4^2*cos(q1)*cos(q2)^2*cos(q3)*sin(q1)*sin(q3))/36893488147419103232 + (d2q2*l3*l4*m4*sin(q3)*sin(q4))/4 + (8907563778312867*dq1*dq4*cos(q1)^2*cos(q2)*sin(q2)*sin(q3))/18446744073709551616 + (8907563778312867*dq2*dq4*cos(q1)*cos(q2)^2*sin(q1)*sin(q3))/18446744073709551616 + (g*l4*m4*cos(q2)*cos(q4)*sin(q1)*sin(q3))/2 - (dq1*dq2*l2*l3*m3*cos(q3)*sin(q2))/2 - dq1*dq2*l2*l3*m4*cos(q3)*sin(q2) - (dq1*dq4*l3*l4*m4*cos(q2)*sin(q4))/2 + (dq2*dq4*l3*l4*m4*cos(q4)*sin(q3))/2 - (dq1*dq4*l4^2*m4*cos(q3)*cos(q4)^2*sin(q2))/4 + (dq1^2*l2*l4*m4*cos(q2)^2*cos(q4)*sin(q3))/4 - (d2q1*l4^2*m4*cos(q3)*cos(q4)*sin(q2)*sin(q4))/8 + (dq1^2*l4^2*m4*cos(q2)^2*cos(q3)*cos(q4)^2*sin(q3))/8 - (1237161635876787*dq1*dq4*cos(q1)*cos(q2)*sin(q1)*sin(q2)*sin(q3))/4611686018427387904 + (d2q1*l2*l4*m4*cos(q2)*cos(q3)*cos(q4))/4 - (d2q1*l3*l4*m4*cos(q3)*sin(q2)*sin(q4))/4 - (dq1*dq2*l4^2*m4*cos(q3)^2*cos(q4)^2*sin(q2))/4 - (dq1*dq4*l4^2*m4*cos(q2)*cos(q4)*sin(q4))/4 + (dq1^2*l1*l4*m4*cos(q2)*cos(q4)*sin(q3))/4 - (dq1^2*l3*l4*m4*cos(q3)*cos(q4)*sin(q3))/2 + (dq2^2*l3*l4*m4*cos(q3)*cos(q4)*sin(q3))/2 + (dq1^2*l3*l4*m4*cos(q2)^2*cos(q3)*cos(q4)*sin(q3))/2 - dq1*dq2*l3*l4*m4*cos(q3)^2*cos(q4)*sin(q2) - (dq1^2*l4^2*m4*cos(q2)*cos(q4)*sin(q2)*sin(q3)*sin(q4))/8 - (dq1*dq2*l4^2*m4*cos(q2)*cos(q3)*cos(q4)*sin(q4))/4 - (dq1^2*l3*l4*m4*cos(q2)*sin(q2)*sin(q3)*sin(q4))/4 - (dq1*dq2*l2*l4*m4*cos(q3)*cos(q4)*sin(q2))/2 - (dq1*dq2*l3*l4*m4*cos(q2)*cos(q3)*sin(q4))/2 - (dq1*dq4*l3*l4*m4*cos(q3)*cos(q4)*sin(q2))/2;
tao4= (6433240506559293*d2q4)/18446744073709551616 + (3958917234805719*d2q2*cos(q3))/18446744073709551616 - (1237161635876787*d2q4*cos(q3)^2)/9223372036854775808 + (5938375852208579*dq2*dq4*sin(q1))/36893488147419103232 - (3958917234805719*dq2*dq3*sin(q3))/18446744073709551616 - (1237161635876787*d2q4*cos(q1)^2*cos(q2)^2)/9223372036854775808 + (1237161635876787*d2q4*cos(q1)^2*cos(q3)^2)/9223372036854775808 + (8907563778312867*dq1*dq4*cos(q2)^2)/36893488147419103232 - (8907563778312867*dq1*dq4*cos(q3)^2)/36893488147419103232 + (1237161635876787*dq3*dq4*sin(2*q3))/9223372036854775808 + (5938375852208579*d2q1*cos(q1)*cos(q3))/73786976294838206464 - (8907563778312867*d2q2*cos(q2)*sin(q3))/73786976294838206464 + (8907563778312867*d2q3*cos(q3)*sin(q2))/73786976294838206464 + (6433240506559293*d2q1*sin(q2)*sin(q3))/18446744073709551616 + (5938375852208579*d2q3*sin(q1)*sin(q3))/73786976294838206464 + (1237161635876787*d2q2*cos(q1)^2*cos(q3))/9223372036854775808 - (5938375852208579*dq1^2*cos(q3)*sin(q1))/73786976294838206464 + (5938375852208579*dq3^2*cos(q3)*sin(q1))/73786976294838206464 + (8907563778312867*dq2^2*sin(q2)*sin(q3))/73786976294838206464 - (8907563778312867*dq3^2*sin(q2)*sin(q3))/73786976294838206464 + (d2q4*l4^2*m4)/8 - (8907563778312867*dq1*dq2*cos(q3))/36893488147419103232 + (8907563778312867*dq3*dq4*cos(q2))/36893488147419103232 - (5938375852208579*dq3^2*cos(q2)^2*cos(q3)*sin(q1))/36893488147419103232 - (8907563778312867*dq2^2*cos(q1)^2*sin(q2)*sin(q3))/36893488147419103232 + (8907563778312867*dq3^2*cos(q1)^2*sin(q2)*sin(q3))/36893488147419103232 + (8907563778312867*dq1*dq2*cos(q1)^2*cos(q3))/18446744073709551616 - (8907563778312867*dq3*dq4*cos(q1)^2*cos(q2))/18446744073709551616 - (8907563778312867*dq3*dq4*cos(q2)*cos(q3)^2)/18446744073709551616 - (1237161635876787*dq2*dq3*cos(q1)^2*sin(q3))/4611686018427387904 - (5938375852208579*dq2*dq4*cos(q2)^2*sin(q1))/18446744073709551616 - (5938375852208579*dq2*dq4*cos(q3)^2*sin(q1))/36893488147419103232 + (5938375852208579*d2q3*cos(q1)*cos(q2)*cos(q3))/73786976294838206464 + (8907563778312867*d2q2*cos(q1)*cos(q3)*sin(q1))/36893488147419103232 - (8907563778312867*d2q4*cos(q2)*cos(q3)*sin(q3))/36893488147419103232 + (1237161635876787*d2q4*cos(q1)^2*cos(q2)^2*cos(q3)^2)/9223372036854775808 - (5938375852208579*d2q1*cos(q2)*sin(q1)*sin(q3))/73786976294838206464 + (5938375852208579*d2q2*cos(q1)*sin(q2)*sin(q3))/73786976294838206464 - (5938375852208579*d2q4*cos(q2)*sin(q1)*sin(q2))/36893488147419103232 - (8907563778312867*dq1*dq4*cos(q1)^2*cos(q2)^2)/18446744073709551616 + (8907563778312867*dq1*dq4*cos(q1)^2*cos(q3)^2)/18446744073709551616 - (8907563778312867*dq1*dq4*cos(q2)^2*cos(q3)^2)/36893488147419103232 - (dq2^2*l4^2*m4*sin(2*q4))/16 + (dq3^2*l4^2*m4*sin(2*q4))/16 + (8907563778312867*d2q2*cos(q1)^2*cos(q2)*sin(q3))/36893488147419103232 - (8907563778312867*d2q4*cos(q1)*cos(q2)^2*sin(q1))/36893488147419103232 - (8907563778312867*d2q3*cos(q1)^2*cos(q3)*sin(q2))/36893488147419103232 + (8907563778312867*d2q4*cos(q1)*cos(q3)^2*sin(q1))/36893488147419103232 - (5938375852208579*dq1^2*cos(q1)*cos(q2)*sin(q3))/73786976294838206464 + (5938375852208579*dq2^2*cos(q1)*cos(q2)*sin(q3))/73786976294838206464 - (5938375852208579*dq3^2*cos(q1)*cos(q2)*sin(q3))/73786976294838206464 - (5938375852208579*d2q3*cos(q2)^2*sin(q1)*sin(q3))/36893488147419103232 + (d2q2*l4^2*m4*cos(q3))/8 + (8907563778312867*dq1*dq2*cos(q2)*sin(q3))/18446744073709551616 + (3958917234805719*dq1*dq3*cos(q3)*sin(q2))/18446744073709551616 - (5938375852208579*dq3*dq4*cos(q1)*sin(q2))/36893488147419103232 - (1237161635876787*dq1*dq2*cos(q1)^2*cos(q2)*sin(q3))/4611686018427387904 + (1237161635876787*dq1*dq4*cos(q1)*cos(q2)^2*sin(q1))/4611686018427387904 - (5938375852208579*dq1*dq3*cos(q1)*cos(q2)^2*sin(q3))/36893488147419103232 + (1237161635876787*dq1*dq3*cos(q1)^2*cos(q3)*sin(q2))/4611686018427387904 - (1237161635876787*dq1*dq4*cos(q1)*cos(q3)^2*sin(q1))/4611686018427387904 + (1237161635876787*dq2*dq4*cos(q1)^2*cos(q2)*sin(q2))/4611686018427387904 + (5938375852208579*dq3*dq4*cos(q1)*cos(q3)^2*sin(q2))/18446744073709551616 - (1237161635876787*dq3*dq4*cos(q1)^2*cos(q3)*sin(q3))/4611686018427387904 - (1237161635876787*d2q2*cos(q1)*cos(q2)*sin(q1)*sin(q3))/9223372036854775808 + (1237161635876787*d2q3*cos(q1)*cos(q3)*sin(q1)*sin(q2))/9223372036854775808 + (5938375852208579*d2q4*cos(q1)*cos(q3)*sin(q2)*sin(q3))/36893488147419103232 + (dq1^2*l3*l4*m4*sin(q4))/4 + (dq3^2*l3*l4*m4*sin(q4))/4 + (8907563778312867*dq3*dq4*cos(q1)^2*cos(q2)*cos(q3)^2)/9223372036854775808 + (1237161635876787*dq2*dq3*cos(q1)^2*cos(q2)^2*sin(q3))/4611686018427387904 + (5938375852208579*dq2*dq4*cos(q2)^2*cos(q3)^2*sin(q1))/18446744073709551616 + (8907563778312867*d2q4*cos(q1)^2*cos(q2)*cos(q3)*sin(q3))/18446744073709551616 + (1237161635876787*d2q3*cos(q1)^2*cos(q2)*sin(q2)*sin(q3))/9223372036854775808 + (5938375852208579*d2q4*cos(q2)*cos(q3)^2*sin(q1)*sin(q2))/36893488147419103232 + (1237161635876787*dq2^2*cos(q1)*sin(q1)*sin(q2)*sin(q3))/9223372036854775808 - (1237161635876787*dq3^2*cos(q1)*sin(q1)*sin(q2)*sin(q3))/9223372036854775808 - (1237161635876787*dq1*dq2*cos(q1)*cos(q3)*sin(q1))/4611686018427387904 - (5938375852208579*dq1*dq3*cos(q2)*cos(q3)*sin(q1))/36893488147419103232 - (5938375852208579*dq1*dq4*cos(q1)*cos(q2)*sin(q2))/36893488147419103232 + (1237161635876787*dq3*dq4*cos(q1)*cos(q2)*sin(q1))/4611686018427387904 + (1237161635876787*dq1*dq4*cos(q2)*cos(q3)*sin(q3))/4611686018427387904 + (8907563778312867*dq1*dq4*cos(q1)^2*cos(q2)^2*cos(q3)^2)/18446744073709551616 + (d2q1*l4^2*m4*sin(q2)*sin(q3))/8 - (8907563778312867*dq2*dq3*cos(q1)*sin(q1)*sin(q3))/18446744073709551616 - (8907563778312867*dq1*dq3*cos(q2)*sin(q2)*sin(q3))/36893488147419103232 + (8907563778312867*dq2*dq4*cos(q3)*sin(q2)*sin(q3))/36893488147419103232 + (d2q2*l2*l4*m4*cos(q4))/4 + (8907563778312867*d2q4*cos(q1)*cos(q2)^2*cos(q3)^2*sin(q1))/36893488147419103232 + (1237161635876787*dq3^2*cos(q1)^2*cos(q2)*cos(q3)*sin(q2))/9223372036854775808 - (1237161635876787*d2q4*cos(q1)*cos(q2)*cos(q3)*sin(q1)*sin(q3))/4611686018427387904 + (8907563778312867*d2q3*cos(q1)*cos(q2)*sin(q1)*sin(q2)*sin(q3))/36893488147419103232 + (dq1*dq2*l4^2*m4*cos(q2)*sin(q3))/4 + (dq1^2*l1*l4*m4*cos(q4)*sin(q2))/4 + (dq2^2*l2*l4*m4*cos(q3)*sin(q4))/4 + (g*l4*m4*cos(q4)*sin(q1)*sin(q2))/2 + (g*l4*m4*cos(q1)*sin(q3)*sin(q4))/2 + (dq1^2*l4^2*m4*cos(q2)^2*cos(q4)*sin(q4))/8 - (dq1^2*l4^2*m4*cos(q3)^2*cos(q4)*sin(q4))/8 + (dq2^2*l4^2*m4*cos(q3)^2*cos(q4)*sin(q4))/8 - (1237161635876787*dq1*dq4*cos(q1)*cos(q2)^2*cos(q3)^2*sin(q1))/4611686018427387904 - (1237161635876787*dq2*dq4*cos(q1)^2*cos(q2)*cos(q3)^2*sin(q2))/4611686018427387904 - (1237161635876787*dq3*dq4*cos(q1)^2*cos(q2)^2*cos(q3)*sin(q3))/4611686018427387904 + (8907563778312867*dq3^2*cos(q1)*cos(q2)*cos(q3)*sin(q1)*sin(q2))/36893488147419103232 - (dq2*dq3*l4^2*m4*cos(q4)^2*sin(q3))/4 - (dq1^2*l3*l4*m4*cos(q3)^2*sin(q4))/4 + (dq2^2*l3*l4*m4*cos(q3)^2*sin(q4))/4 + (5938375852208579*dq2*dq4*cos(q1)*cos(q2)*cos(q3)*sin(q3))/36893488147419103232 - (8907563778312867*dq1*dq2*cos(q1)*cos(q2)*sin(q1)*sin(q3))/18446744073709551616 + (8907563778312867*dq1*dq3*cos(q1)*cos(q3)*sin(q1)*sin(q2))/18446744073709551616 + (8907563778312867*dq2*dq4*cos(q1)*cos(q2)*sin(q1)*sin(q2))/18446744073709551616 - (8907563778312867*dq3*dq4*cos(q1)*cos(q3)*sin(q1)*sin(q3))/18446744073709551616 + (5938375852208579*dq2*dq3*cos(q2)*sin(q1)*sin(q2)*sin(q3))/18446744073709551616 - (5938375852208579*dq1*dq4*cos(q3)*sin(q1)*sin(q2)*sin(q3))/36893488147419103232 + (d2q2*l3*l4*m4*cos(q3)*cos(q4))/4 - (d2q1*l1*l4*m4*sin(q3)*sin(q4))/4 - (dq1^2*l4^2*m4*cos(q2)*cos(q3)*sin(q2))/8 + (5938375852208579*dq1*dq4*cos(q1)*cos(q2)*cos(q3)^2*sin(q2))/36893488147419103232 - (1237161635876787*dq1*dq4*cos(q1)^2*cos(q2)*cos(q3)*sin(q3))/2305843009213693952 - (1237161635876787*dq3*dq4*cos(q1)*cos(q2)*cos(q3)^2*sin(q1))/2305843009213693952 + (8907563778312867*dq1*dq3*cos(q1)^2*cos(q2)*sin(q2)*sin(q3))/18446744073709551616 + (8907563778312867*dq2*dq3*cos(q1)*cos(q2)^2*sin(q1)*sin(q3))/18446744073709551616 - (8907563778312867*dq2*dq4*cos(q1)^2*cos(q3)*sin(q2)*sin(q3))/18446744073709551616 + (g*l4*m4*cos(q2)*cos(q3)*sin(q1)*sin(q4))/2 + (dq1^2*l4^2*m4*cos(q2)*cos(q3)*cos(q4)^2*sin(q2))/4 + (dq1*dq3*l3*l4*m4*cos(q2)*sin(q4))/2 - (dq2*dq3*l3*l4*m4*cos(q4)*sin(q3))/2 - (dq1*dq2*l4^2*m4*cos(q2)*cos(q4)^2*sin(q3))/4 + (dq1*dq3*l4^2*m4*cos(q3)*cos(q4)^2*sin(q2))/4 + (dq1^2*l2*l4*m4*cos(q2)^2*cos(q3)*sin(q4))/4 - (8907563778312867*dq1*dq4*cos(q1)*cos(q2)*cos(q3)*sin(q1)*sin(q3))/9223372036854775808 + (dq1^2*l4^2*m4*cos(q2)^2*cos(q3)^2*cos(q4)*sin(q4))/8 - (1237161635876787*dq1*dq3*cos(q1)*cos(q2)*sin(q1)*sin(q2)*sin(q3))/4611686018427387904 + (1237161635876787*dq2*dq4*cos(q1)*cos(q3)*sin(q1)*sin(q2)*sin(q3))/4611686018427387904 - (5938375852208579*dq3*dq4*cos(q2)*cos(q3)*sin(q1)*sin(q2)*sin(q3))/18446744073709551616 - (d2q1*l2*l4*m4*cos(q2)*sin(q3)*sin(q4))/4 + (d2q1*l3*l4*m4*cos(q4)*sin(q2)*sin(q3))/4 + (dq1^2*l3*l4*m4*cos(q2)^2*cos(q3)^2*sin(q4))/4 - (8907563778312867*dq2*dq4*cos(q1)*cos(q2)*cos(q3)^2*sin(q1)*sin(q2))/18446744073709551616 - (8907563778312867*dq3*dq4*cos(q1)*cos(q2)^2*cos(q3)*sin(q1)*sin(q3))/18446744073709551616 + (dq1*dq3*l4^2*m4*cos(q2)*cos(q4)*sin(q4))/4 + (dq1^2*l1*l4*m4*cos(q2)*cos(q3)*sin(q4))/4 + (dq1^2*l2*l4*m4*cos(q2)*cos(q4)*sin(q2))/4 + (dq1*dq2*l2*l4*m4*sin(q2)*sin(q3)*sin(q4))/2 + (dq1^2*l3*l4*m4*cos(q2)*cos(q3)*cos(q4)*sin(q2))/4 + (dq1*dq3*l3*l4*m4*cos(q3)*cos(q4)*sin(q2))/2 + (dq1*dq2*l4^2*m4*cos(q3)*cos(q4)*sin(q2)*sin(q3)*sin(q4))/4 + (dq1*dq2*l3*l4*m4*cos(q3)*sin(q2)*sin(q3)*sin(q4))/2;
end
